simulink model "Copter_Plane_h2g_V10"  (R2020b)
settings: Solver=ode1  StartTime=0.0  StopTime=30  FixedStep=dt  RelTol=1e-3
values from neighbouring files (symbols this model uses):
  HD = 180/pi    (= 57.2957795131)    [mode_data.m]
undefined symbols (not defined in the file or in its folder): center_WP, GRAVITY_MSS, gyro_x, gyro_y, gyro_z, J, k_aileron, k_aileronL, k_aileronR, k_elevator, k_flap, k_rudder, m_kg, Newton, pid_vel_xy_derivative, pid_vel_xy_input, pid_vel_xy_integrator, pitch, POSCONTROL_ACC_Z_D, POSCONTROL_ACC_Z_P, POSCONTROL_VEL_XY_D, POSCONTROL_VEL_XY_P, pwm_out, pwm_tail, Raphson, roll, tail_tilt, Vehicle, vel_desired, yaw
libraries: shared6dofsys x3, sharedutil x3, simulink x1, aerolibasang x1
(part 2 of 3)

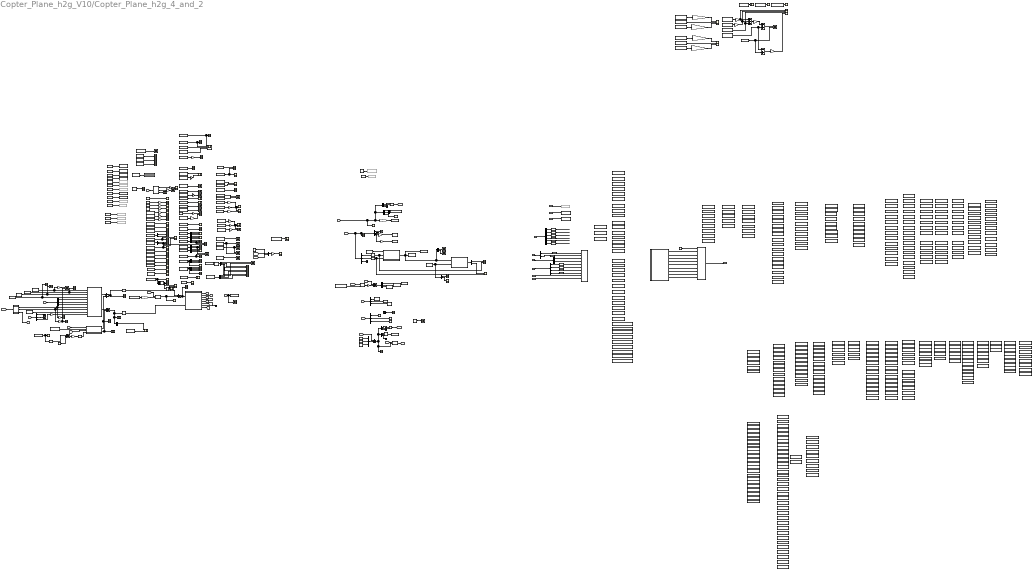
== system Copter_Plane_h2g_V10/Copter_Plane_h2g_4_and_2 ==
  CTRL_wp : Inport
  CTRL_remote_ct_st : Inport  Port=2  OutDataTypeStr=Bus: BUS_CTRL_remote_ct_st
  CTRL_dbg_param : Inport  Port=3  OutDataTypeStr=Bus: BUS_CTRL_dbg_param
  PathModeOut : Inport  Port=4  OutDataTypeStr=Bus: BUS_TASK_PATH_OutParam
  TASK_COMMON_OutParam : Inport  Port=5  OutDataTypeStr=Bus: BUS_TASK_COMMON_OutParam
  NAVI2CONTROL : Inport  Port=6  OutDataTypeStr=Bus: BUS_TO_CONTROL
  EAS_Algo : Inport  Port=7  OutDataTypeStr=Bus: BUS_AIRSPEED
  IMU : Inport  Port=8  OutDataTypeStr=Bus: BUS_IMU
  plane_mode_in : Inport  Port=9
  6DOF (Euler Angles)2 : Subsystem  AncestorBlock=shared6dof/6DOF (Euler Angles)  mask(6DOF EoM (Body Axis)){units=Metric (MKS), mtype=Fixed, rep=Euler Angles, xme_0=[0 0 -100], Vm_0=[10 -0 0], eul_0=[roll pitch yaw], pm_0=[gyro_x gyro_y gyro_z], mass_0=m_kg, mass_e=0.5, mass_f=2.0, inertia=J, inertia_e=eye(3), inertia_f=2*eye(3), k_quat=1.0, vre_flag=on, abi_flag=off, aMode=0, xme_statename='', Vm_statename='', eul_statename='', quat_statename='', pm_statename='', mass_statename=''}
      mask prompts: units "shared_aeroblks:sharedaeroblk6dofbody:block6DOFEoMBodyAxisParamUnits"; mtype "shared_aeroblks:sharedaeroblk6dofbody:block6DOFEoMBodyAxisParamMasstype"; rep "shared_aeroblks:sharedaeroblk6dofbody:block6DOFEoMBodyAxisParamRepresentation"; xme_0 "shared_aeroblks:sharedaeroblk6dofbody:block6DOFEoMBodyAxisParamInitialpositionininertialaxesXeYeZe"; Vm_0 "shared_aeroblks:sharedaeroblk6dofbody:block6DOFEoMBodyAxisParamInitialvelocityinbodyaxesUvw"; eul_0 "shared_aeroblks:sharedaeroblk6dofbody:block6DOFEoMBodyAxisParamInitialEulerorientationrollpitchyaw"; pm_0 "shared_aeroblks:sharedaeroblk6dofbody:block6DOFEoMBodyAxisParamInitialbodyrotationratespqr"; mass_0 "shared_aeroblks:sharedaeroblk6dofbody:block6DOFEoMBodyAxisParamInitialmass"; mass_e "shared_aeroblks:sharedaeroblk6dofbody:block6DOFEoMBodyAxisParamEmptymass"; mass_f "shared_aeroblks:sharedaeroblk6dofbody:block6DOFEoMBodyAxisParamFullmass"; inertia "shared_aeroblks:sharedaeroblk6dofbody:block6DOFEoMBodyAxisParamInertia"; inertia_e "shared_aeroblks:sharedaeroblk6dofbody:block6DOFEoMBodyAxisParamEmptyinertiamatrix"; inertia_f "shared_aeroblks:sharedaeroblk6dofbody:block6DOFEoMBodyAxisParamFullinertiamatrix"; k_quat "shared_aeroblks:sharedaeroblk6dofbody:block6DOFEoMBodyAxisParamGainforquaternionnormalization"; vre_flag "shared_aeroblks:sharedaeroblk6dofbody:block6DOFEoMBodyAxisParamIncludemassflowrelativevelocity"; abi_flag "shared_aeroblks:sharedaeroblk6dofbody:inertialAccelFlag"; xme_statename "shared_aeroblks:sharedaeroblk6dofbody:block6DOFEoMStateNamePosition"; Vm_statename "shared_aeroblks:sharedaeroblk6dofbody:block6DOFEoMStateNameVelocity"; eul_statename "shared_aeroblks:sharedaeroblk6dofbody:block6DOFEoMStateNameEulerAngles"; quat_statename "shared_aeroblks:sharedaeroblk6dofbody:block6DOFEoMStateNameQuaternions"; pm_statename "shared_aeroblks:sharedaeroblk6dofbody:block6DOFEoMStateNameRotationRates"; mass_statename "shared_aeroblks:sharedaeroblk6dofbody:block6DOFEoMStateNameMass"
      mask help: shared_aeroblks:sharedaeroblk6dofbody:block6DOFEoMBodyAxisDesc
      mask init:
      | if aerosharedtest(gcb)
      |     ports=aerosharedicon('shared6dofbody','icon');
      | else
      |     ports=sharedautoicon('shared6dofbody','icon');
      | end
      mask Help: eval('aerosharedhelp(''sixdof_euler_angles'')');
      mask TypeOptions units: shared_aeroblks:sharedaeroblk6dofbody:block6DOFEoMBodyAxisParamComboMetricMKS | shared_aeroblks:sharedaeroblk6dofbody:block6DOFEoMBodyAxisParamComboEnglishVelocityinfts | shared_aeroblks:sharedaeroblk6dofbody:block6DOFEoMBodyAxisParamComboEnglishVelocityinkts
      mask TypeOptions mtype: shared_aeroblks:sharedaeroblk6dofbody:block6DOFEoMBodyAxisParamComboFixed | shared_aeroblks:sharedaeroblk6dofbody:block6DOFEoMBodyAxisParamComboSimpleVariable | shared_aeroblks:sharedaeroblk6dofbody:block6DOFEoMBodyAxisParamComboCustomVariable
      mask Callback mtype:
      | if aerosharedtest(gcb) && builtin('license','test','aerospace_blockset')
      |     aerosharedicon('shared6dofbody');
      | else
      |     sharedautoicon('shared6dofbody');
      | end
      mask TypeOptions rep: shared_aeroblks:sharedaeroblk6dofbody:block6DOFEoMBodyAxisParamComboEulerAngles | shared_aeroblks:sharedaeroblk6dofbody:block6DOFEoMBodyAxisParamComboQuaternion
      mask Callback rep:
      | if aerosharedtest(gcb) && builtin('license','test','aerospace_blockset')
      |     aerosharedicon('shared6dofbody');
      | else
      |     sharedautoicon('shared6dofbody');
      | end
      mask DialogControl Container4 Prompt: shared_aeroblks:sharedaeroblk6dofbody:block6DOFEoMParamTab
      mask DialogControl units Prompt: Units:
      mask DialogControl mtype Prompt: Mass type:
      mask DialogControl rep Prompt: Representation:
      mask DialogControl xme_0 Prompt: Initial position in inertial axes [Xe,Ye,Ze]:
      mask DialogControl Vm_0 Prompt: Initial velocity in body axes [U,v,w]:
      mask DialogControl eul_0 Prompt: Initial Euler orientation [roll, pitch, yaw]:
      mask DialogControl pm_0 Prompt: Initial body rotation rates [p,q,r]:
      mask DialogControl mass_0 Prompt: Initial mass:
      mask DialogControl mass_e Prompt: Empty mass:
      mask DialogControl mass_f Prompt: Full mass:
      mask DialogControl inertia Prompt: Inertia:
      mask DialogControl inertia_e Prompt: Empty inertia matrix:
      mask DialogControl inertia_f Prompt: Full inertia matrix:
      mask DialogControl k_quat Prompt: Gain for quaternion normalization:
      mask DialogControl vre_flag Prompt: Include mass flow relative velocity
      mask DialogControl abi_flag Prompt: Include inertial acceleration
      mask DialogControl Container6 Prompt: shared_aeroblks:sharedaeroblk6dofbody:block6DOFEoMStateAttributesTab
      mask DialogControl Container7 Prompt: shared_aeroblks:sharedaeroblk6dofbody:block6DOFEoMStateNamesGroup
      mask DialogControl xme_statename Prompt: Position: e.g., {'Xe', 'Ye', 'Ze'}
      mask DialogControl Vm_statename Prompt: Velocity: e.g., {'U', 'v', 'w'}
      mask DialogControl eul_statename Prompt: Euler rotation angles: e.g., {'phi', 'theta', 'psi'}
      mask DialogControl quat_statename Prompt: Quaternion vector: e.g., {'qr', 'qi', 'qj', 'qk'}
      mask DialogControl pm_statename Prompt: Body rotation rates: e.g., {'p', 'q', 'r'}
      mask DialogControl mass_statename Prompt: Mass: e.g., 'mass'
      mask Display:
      | port_label(ports(1).type,ports(1).port,ports(1).txt,'texmode','on');
      | port_label(ports(2).type,ports(2).port,ports(2).txt,'texmode','on');
      | port_label(ports(3).type,ports(3).port,ports(3).txt,'texmode','on');
      | port_label(ports(4).type,ports(4).port,ports(4).txt,'texmode','on');
      | port_label(ports(5).type,ports(5).port,ports(5).txt,'texmode','on');
      | port_label(ports(6).type,ports(6).port,ports(6).txt,'texmode','on');
      | port_label(ports(7).type,ports(7).port,ports(7).txt,'texmode','on');
      | port_label(ports(8).type,ports(8).port,ports(8).txt,'texmode','on');
      | port_label(ports(9).type,ports(9).port,ports(9).txt,'texmode','on');
      | port_label(ports(10).type,ports(10).port,ports(10).txt,'texmode','on');
      | port_label(ports(11).type,ports(11).port,ports(11).txt,'texmode','on');
      | port_label(ports(12).type,ports(12).port,ports(12).txt,'texmode','on');
      | port_label(ports(13).type,ports(13).port,ports(13).txt,'texmode','on');
      | port_label(ports(14).type,ports(14).port,ports(14).txt,'texmode','on');
      | port_label(ports(15).type,ports(15).port,ports(15).txt,'texmode','on');
      | port_label(ports(16).type,ports(16).port,ports(16).txt,'texmode','on');
      | port_label(ports(17).type,ports(17).port,ports(17).txt,'texmode','on');
  AC_ATTITUDE_ACCEL_RP_CONTROLLER_MAX_RADSS1 : DataStoreMemory  DataStoreName=AC_ATTITUDE_ACCEL_RP_CONTROLLER_MAX_RADSS  ReadBeforeWriteMsg=warning  WriteAfterWriteMsg=warning  WriteAfterReadMsg=warning  InitialValue=AC_ATTITUDE_ACCEL_RP_CONTROLLER_MAX_RADSS  VectorParams1D=off  ShowAdditionalParam=off  OutDataTypeStr=double
  AC_ATTITUDE_ACCEL_RP_CONTROLLER_MIN_RADSS1 : DataStoreMemory  DataStoreName=AC_ATTITUDE_ACCEL_RP_CONTROLLER_MIN_RADSS  ReadBeforeWriteMsg=warning  WriteAfterWriteMsg=warning  WriteAfterReadMsg=warning  InitialValue=AC_ATTITUDE_ACCEL_RP_CONTROLLER_MIN_RADSS  VectorParams1D=off  ShowAdditionalParam=off  OutDataTypeStr=double
  AC_ATTITUDE_ACCEL_Y_CONTROLLER_MAX_RADSS1 : DataStoreMemory  DataStoreName=AC_ATTITUDE_ACCEL_Y_CONTROLLER_MAX_RADSS  ReadBeforeWriteMsg=warning  WriteAfterWriteMsg=warning  WriteAfterReadMsg=warning  InitialValue=AC_ATTITUDE_ACCEL_Y_CONTROLLER_MAX_RADSS  ShowAdditionalParam=off  OutDataTypeStr=double
  AC_ATTITUDE_ACCEL_Y_CONTROLLER_MIN_RADSS1 : DataStoreMemory  DataStoreName=AC_ATTITUDE_ACCEL_Y_CONTROLLER_MIN_RADSS  ReadBeforeWriteMsg=warning  WriteAfterWriteMsg=warning  WriteAfterReadMsg=warning  InitialValue=AC_ATTITUDE_ACCEL_Y_CONTROLLER_MIN_RADSS  VectorParams1D=off  ShowAdditionalParam=off  OutDataTypeStr=double
  AC_ATTITUDE_CONTROL_ANGLE_LIMIT_THROTTLE_MAX1 : DataStoreMemory  DataStoreName=AC_ATTITUDE_CONTROL_ANGLE_LIMIT_THROTTLE_MAX  ReadBeforeWriteMsg=warning  WriteAfterWriteMsg=warning  WriteAfterReadMsg=warning  InitialValue=AC_ATTITUDE_CONTROL_ANGLE_LIMIT_THROTTLE_MAX  VectorParams1D=off  ShowAdditionalParam=off  OutDataTypeStr=double
  AC_ATTITUDE_CONTROL_MAX1 : DataStoreMemory  DataStoreName=AC_ATTITUDE_CONTROL_MAX  ReadBeforeWriteMsg=warning  WriteAfterWriteMsg=warning  WriteAfterReadMsg=warning  InitialValue=AC_ATTITUDE_CONTROL_MAX  VectorParams1D=off  ShowAdditionalParam=off  OutDataTypeStr=double
  AC_ATTITUDE_THRUST_ERROR_ANGLE1 : DataStoreMemory  DataStoreName=AC_ATTITUDE_THRUST_ERROR_ANGLE  ReadBeforeWriteMsg=warning  WriteAfterWriteMsg=warning  WriteAfterReadMsg=warning  InitialValue=AC_ATTITUDE_THRUST_ERROR_ANGLE  ShowAdditionalParam=off  OutDataTypeStr=double
  AP_MOTORS_MATRIX_YAW_FACTOR_CCW1 : DataStoreMemory  DataStoreName=AP_MOTORS_MATRIX_YAW_FACTOR_CCW  ReadBeforeWriteMsg=warning  WriteAfterWriteMsg=warning  WriteAfterReadMsg=warning  InitialValue=AP_MOTORS_MATRIX_YAW_FACTOR_CCW  VectorParams1D=off  ShowAdditionalParam=off  OutDataTypeStr=double
  AP_MOTORS_MATRIX_YAW_FACTOR_CW1 : DataStoreMemory  DataStoreName=AP_MOTORS_MATRIX_YAW_FACTOR_CW  ReadBeforeWriteMsg=warning  WriteAfterWriteMsg=warning  WriteAfterReadMsg=warning  InitialValue=AP_MOTORS_MATRIX_YAW_FACTOR_CW  VectorParams1D=off  ShowAdditionalParam=off  OutDataTypeStr=double
  ATC_RAT_PIT_D1 : DataStoreMemory  DataStoreName=ATC_RAT_PIT_D  ReadBeforeWriteMsg=warning  WriteAfterWriteMsg=warning  WriteAfterReadMsg=warning  InitialValue=ATC_RAT_PIT_D  VectorParams1D=off  ShowAdditionalParam=off  OutDataTypeStr=double
  ATC_RAT_PIT_FF1 : DataStoreMemory  DataStoreName=ATC_RAT_PIT_FF  ReadBeforeWriteMsg=warning  WriteAfterWriteMsg=warning  WriteAfterReadMsg=warning  InitialValue=ATC_RAT_PIT_FF  VectorParams1D=off  ShowAdditionalParam=off  OutDataTypeStr=double
  ATC_RAT_PIT_FILT1 : DataStoreMemory  DataStoreName=ATC_RAT_PIT_FILT  ReadBeforeWriteMsg=warning  WriteAfterWriteMsg=warning  WriteAfterReadMsg=warning  InitialValue=ATC_RAT_PIT_FILT  VectorParams1D=off  ShowAdditionalParam=off  OutDataTypeStr=double
  ATC_RAT_PIT_I1 : DataStoreMemory  DataStoreName=ATC_RAT_PIT_I  ReadBeforeWriteMsg=warning  WriteAfterWriteMsg=warning  WriteAfterReadMsg=warning  InitialValue=ATC_RAT_PIT_I  VectorParams1D=off  ShowAdditionalParam=off  OutDataTypeStr=double
  ATC_RAT_PIT_IMAX1 : DataStoreMemory  DataStoreName=ATC_RAT_PIT_IMAX  ReadBeforeWriteMsg=warning  WriteAfterWriteMsg=warning  WriteAfterReadMsg=warning  InitialValue=ATC_RAT_PIT_IMAX  VectorParams1D=off  ShowAdditionalParam=off  OutDataTypeStr=double
  ATC_RAT_PIT_I_inint1 : DataStoreMemory  DataStoreName=ATC_RAT_PIT_I_inint  ReadBeforeWriteMsg=warning  WriteAfterWriteMsg=warning  WriteAfterReadMsg=warning  InitialValue=ATC_RAT_PIT_I_inint  VectorParams1D=off  ShowAdditionalParam=off  OutDataTypeStr=double
  ATC_RAT_PIT_P1 : DataStoreMemory  DataStoreName=ATC_RAT_PIT_P  ReadBeforeWriteMsg=warning  WriteAfterWriteMsg=warning  WriteAfterReadMsg=warning  InitialValue=ATC_RAT_PIT_P  VectorParams1D=off  ShowAdditionalParam=off  OutDataTypeStr=double
  ATC_RAT_RLL_D1 : DataStoreMemory  DataStoreName=ATC_RAT_RLL_D  ReadBeforeWriteMsg=warning  WriteAfterWriteMsg=warning  WriteAfterReadMsg=warning  InitialValue=ATC_RAT_RLL_D  VectorParams1D=off  ShowAdditionalParam=off  OutDataTypeStr=double
  ATC_RAT_RLL_FF1 : DataStoreMemory  DataStoreName=ATC_RAT_RLL_FF  ReadBeforeWriteMsg=warning  WriteAfterWriteMsg=warning  WriteAfterReadMsg=warning  InitialValue=ATC_RAT_RLL_FF  VectorParams1D=off  ShowAdditionalParam=off  OutDataTypeStr=double
  ATC_RAT_RLL_FILT1 : DataStoreMemory  DataStoreName=ATC_RAT_RLL_FILT  ReadBeforeWriteMsg=warning  WriteAfterWriteMsg=warning  WriteAfterReadMsg=warning  InitialValue=ATC_RAT_RLL_FILT  VectorParams1D=off  ShowAdditionalParam=off  OutDataTypeStr=double
  ATC_RAT_RLL_I1 : DataStoreMemory  DataStoreName=ATC_RAT_RLL_I  ReadBeforeWriteMsg=warning  WriteAfterWriteMsg=warning  WriteAfterReadMsg=warning  InitialValue=ATC_RAT_RLL_I  VectorParams1D=off  ShowAdditionalParam=off  OutDataTypeStr=double
  ATC_RAT_RLL_IMAX1 : DataStoreMemory  DataStoreName=ATC_RAT_RLL_IMAX  ReadBeforeWriteMsg=warning  WriteAfterWriteMsg=warning  WriteAfterReadMsg=warning  InitialValue=ATC_RAT_RLL_IMAX  VectorParams1D=off  ShowAdditionalParam=off  OutDataTypeStr=double
  ATC_RAT_RLL_I_inint1 : DataStoreMemory  DataStoreName=ATC_RAT_RLL_I_inint  ReadBeforeWriteMsg=warning  WriteAfterWriteMsg=warning  WriteAfterReadMsg=warning  InitialValue=ATC_RAT_RLL_I_inint  VectorParams1D=off  ShowAdditionalParam=off  OutDataTypeStr=double
  ATC_RAT_RLL_P1 : DataStoreMemory  DataStoreName=ATC_RAT_RLL_P  ReadBeforeWriteMsg=warning  WriteAfterWriteMsg=warning  WriteAfterReadMsg=warning  InitialValue=ATC_RAT_RLL_P  VectorParams1D=off  ShowAdditionalParam=off  OutDataTypeStr=double
  ATC_RAT_YAW_D1 : DataStoreMemory  DataStoreName=ATC_RAT_YAW_D  ReadBeforeWriteMsg=warning  WriteAfterWriteMsg=warning  WriteAfterReadMsg=warning  InitialValue=ATC_RAT_YAW_D  VectorParams1D=off  ShowAdditionalParam=off  OutDataTypeStr=double
  ATC_RAT_YAW_FF1 : DataStoreMemory  DataStoreName=ATC_RAT_YAW_FF  ReadBeforeWriteMsg=warning  WriteAfterWriteMsg=warning  WriteAfterReadMsg=warning  InitialValue=ATC_RAT_YAW_FF  VectorParams1D=off  ShowAdditionalParam=off  OutDataTypeStr=double
  ATC_RAT_YAW_FILT1 : DataStoreMemory  DataStoreName=ATC_RAT_YAW_FILT  ReadBeforeWriteMsg=warning  WriteAfterWriteMsg=warning  WriteAfterReadMsg=warning  InitialValue=ATC_RAT_YAW_FILT  VectorParams1D=off  ShowAdditionalParam=off  OutDataTypeStr=double
  ATC_RAT_YAW_I1 : DataStoreMemory  DataStoreName=ATC_RAT_YAW_I  ReadBeforeWriteMsg=warning  WriteAfterWriteMsg=warning  WriteAfterReadMsg=warning  InitialValue=ATC_RAT_YAW_I  VectorParams1D=off  ShowAdditionalParam=off  OutDataTypeStr=double
  ATC_RAT_YAW_IMAX1 : DataStoreMemory  DataStoreName=ATC_RAT_YAW_IMAX  ReadBeforeWriteMsg=warning  WriteAfterWriteMsg=warning  WriteAfterReadMsg=warning  InitialValue=ATC_RAT_YAW_IMAX  VectorParams1D=off  ShowAdditionalParam=off  OutDataTypeStr=double
  ATC_RAT_YAW_I_inint1 : DataStoreMemory  DataStoreName=ATC_RAT_YAW_I_inint  ReadBeforeWriteMsg=warning  WriteAfterWriteMsg=warning  WriteAfterReadMsg=warning  InitialValue=ATC_RAT_YAW_I_inint  VectorParams1D=off  ShowAdditionalParam=off  OutDataTypeStr=double
  ATC_RAT_YAW_P1 : DataStoreMemory  DataStoreName=ATC_RAT_YAW_P  ReadBeforeWriteMsg=warning  WriteAfterWriteMsg=warning  WriteAfterReadMsg=warning  InitialValue=ATC_RAT_YAW_P  VectorParams1D=off  ShowAdditionalParam=off  OutDataTypeStr=double
  Add : Sum  Inputs=+++
  Add{1..3,5,7} (5 alike) : Sum
  Add4 : Sum  Inputs=-+
  Add8 : Sum  Inputs=+-
  Atan3 : Trigonometry  Operator=atan2
  Atan4 : Trigonometry  Operator=atan2
  Bus Assignment : BusAssignment  AssignedSignals=k_aileron,k_elevator,k_rudder,k_aileronL,k_aileronR,tail_tilt,pwm_out,pwm_tail,k_flap
  Bus Selector : BusSelector  OutputSignals=curVelNED,curLLA
  Bus Selector1 : BusSelector  OutputSignals=pitchd,rolld,yawd,alt
  Bus Selector2 : BusSelector  OutputSignals=gyro_x,gyro_y,gyro_z,accel_x,accel_y,accel_z
  Bus Selector3 : BusSelector  OutputSignals=airspeed_indicate,EAS2TAS_Algo
  Constant : Constant  Value=0  OutDataTypeStr=Bus: BUS_CTRL_Sevro_pwm
  Constant1 : Constant  Value=0.3
  Constant{12..14,26,30,33,37,40..41} (9 alike) : Constant  Value=0
  Constant2 : Constant  Value=1000  VectorParams1D=off
  Constant25 : Constant  Value=500
  Constant27 : Constant  Value=10
  Constant28 : Constant  Value=500
  Constant29 : Constant  Value=000
  Constant31 : Constant  Value=[0;0]
  Constant32 : Constant  Value=0/HD
  Constant34 : Constant  Value=0.25
  Constant35 : Constant  Value=0.3
  Constant36 : Constant  Value=center_WP
  Constant38 : Constant  Value=center_WP
  Constant39 : Constant  Value=-30/HD
  Constant5 : Constant  Value=1.225
  Curr_sate : DataStoreMemory  DataStoreName=Curr_sate  ReadBeforeWriteMsg=warning  WriteAfterWriteMsg=warning  WriteAfterReadMsg=warning  InitialValue=Curr_sate  VectorParams1D=off  ShowAdditionalParam=off  OutDataTypeStr=Bus: BUS_CTRL_Curr_sate
  Data Store Read : DataStoreRead  DataStoreName=pitch_target
  Data Store Read1 : DataStoreRead  DataStoreName=pid_info_P_pitch
  Data Store Read10 : DataStoreRead  DataStoreName=pid_accel_z_integrator
  Data Store Read107 : DataStoreRead  DataStoreName=gyro_y
  Data Store Read108 : DataStoreRead  DataStoreName=curr_pos
  Data Store Read109 : DataStoreRead  DataStoreName=curr_alt
  Data Store Read11 : DataStoreRead  DataStoreName=pid_accel_z_input
  Data Store Read110 : DataStoreRead  DataStoreName=nav_bearing
  Data Store Read111 : DataStoreRead  DataStoreName=k_rudder
  Data Store Read112 : DataStoreRead  DataStoreName=k_aileron
  Data Store Read113 : DataStoreRead  DataStoreName=mode_L1
  Data Store Read114 : DataStoreRead  DataStoreName=k_throttle
  Data Store Read116 : DataStoreRead  DataStoreName=k_elevator
  Data Store Read117 : DataStoreRead  DataStoreName=roll
  Data Store Read118 : DataStoreRead  DataStoreName=pitch
  Data Store Read119 : DataStoreRead  DataStoreName=yaw
  Data Store Read12 : DataStoreRead  DataStoreName=pwm_out
  Data Store Read120 : DataStoreRead  DataStoreName=curr_vel
  Data Store Read121 : DataStoreRead  DataStoreName=z_accel_meas
  Data Store Read122 : DataStoreRead  DataStoreName=latAccDem
  Data Store Read123 : DataStoreRead  DataStoreName=accel_x
  Data Store Read124 : DataStoreRead  DataStoreName=accel_y
  Data Store Read125 : DataStoreRead  DataStoreName=accel_z
  Data Store Read126 : DataStoreRead  DataStoreName=pwm_out
  Data Store Read127 : DataStoreRead  DataStoreName=pos_target
  Data Store Read128 : DataStoreRead  DataStoreName=vel_target
  Data Store Read129 : DataStoreRead  DataStoreName=vel_desired
  Data Store Read13 : DataStoreRead  DataStoreName=thrust_rpyt_out
  Data Store Read130 : DataStoreRead  DataStoreName=accel_target
  Data Store Read131 : DataStoreRead  DataStoreName=accel_desired
  Data Store Read132 : DataStoreRead  DataStoreName=throttle_filter
  Data Store Read133 : DataStoreRead  DataStoreName=EAS_dem
  Data Store Read134 : DataStoreRead  DataStoreName=nav_pitch_cd
  Data Store Read135 : DataStoreRead  DataStoreName=aspeed
  Data Store Read136 : DataStoreRead  DataStoreName=nav_roll_cd
  Data Store Read137 : DataStoreRead  DataStoreName=k_rudder
  Data Store Read138 : DataStoreRead  DataStoreName=k_aileron
  Data Store Read139 : DataStoreRead  DataStoreName=k_throttle
  Data Store Read14 : DataStoreRead  DataStoreName=pitch_in
  Data Store Read140 : DataStoreRead  DataStoreName=k_elevator
  Data Store Read141 : DataStoreRead  DataStoreName=height
  Data Store Read142 : DataStoreRead  DataStoreName=Vz
  Data Store Read143 : DataStoreRead  DataStoreName=roll
  Data Store Read144 : DataStoreRead  DataStoreName=pid_vel_xy_input  DataStoreElements=pid_vel_xy_input(:,1)
  Data Store Read145 : DataStoreRead  DataStoreName=pid_vel_xy_integrator  DataStoreElements=pid_vel_xy_integrator(:,1)
  Data Store Read146 : DataStoreRead  DataStoreName=pid_vel_xy_derivative  DataStoreElements=pid_vel_xy_derivative(:,1)
  Data Store Read147 : DataStoreRead  DataStoreName=pid_vel_xy_input  DataStoreElements=pid_vel_xy_input(:,2)
  Data Store Read148 : DataStoreRead  DataStoreName=pid_vel_xy_integrator  DataStoreElements=pid_vel_xy_integrator(:,2)
  Data Store Read149 : DataStoreRead  DataStoreName=pid_vel_xy_derivative  DataStoreElements=pid_vel_xy_derivative(:,2)
  Data Store Read15 : DataStoreRead  DataStoreName=k_flap
  Data Store Read150 : DataStoreRead  DataStoreName=pid_info_I_pitch
  Data Store Read151 : DataStoreRead  DataStoreName=last_out_pitch
  Data Store Read16 : DataStoreRead  DataStoreName=aspeed
  Data Store Read166 : DataStoreRead  DataStoreName=throttle_hover
  Data Store Read167 : DataStoreRead  DataStoreName=throttle_in
  Data Store Read17 : DataStoreRead  DataStoreName=pwm_out
  Data Store Read18 : DataStoreRead  DataStoreName=plane_mode
  Data Store Read2 : DataStoreRead  DataStoreName=k_flap_Land
  Data Store Read3 : DataStoreRead  DataStoreName=k_flap_TakeOff
  Data Store Read34 : DataStoreRead  DataStoreName=hgt_rate_dem
  Data Store Read36 : DataStoreRead  DataStoreName=nav_roll_cd
  Data Store Read37 : DataStoreRead  DataStoreName=throttle_dem
  Data Store Read38 : DataStoreRead  DataStoreName=pitch_dem
  Data Store Read39 : DataStoreRead  DataStoreName=nav_pitch_cd
  Data Store Read4 : DataStoreRead  DataStoreName=rate_roll_pid_integrator
  Data Store Read40 : DataStoreRead  DataStoreName=pitch
  Data Store Read41 : DataStoreRead  DataStoreName=pid_info_desired_pitch
  Data Store Read42 : DataStoreRead  DataStoreName=pid_info_actual_pitch
  Data Store Read43 : DataStoreRead  DataStoreName=hgt_dem_adj
  Data Store Read44 : DataStoreRead  DataStoreName=height
  Data Store Read45 : DataStoreRead  DataStoreName=hgt_dem_adj
  Data Store Read46 : DataStoreRead  DataStoreName=Vz
  Data Store Read48 : DataStoreRead  DataStoreName=thrust_rpyt_out
  Data Store Read5 : DataStoreRead  DataStoreName=rate_pitch_pid_integrator
  Data Store Read50 : DataStoreRead  DataStoreName=pitch_in
  Data Store Read53 : DataStoreRead  DataStoreName=pitch_target
  Data Store Read54 : DataStoreRead  DataStoreName=roll_target
  Data Store Read55 : DataStoreRead  DataStoreName=target_yaw_rate
  Data Store Read56 : DataStoreRead  DataStoreName=mode
  Data Store Read57 : DataStoreRead  DataStoreName=tail_tilt
  Data Store Read58 : DataStoreRead  DataStoreName=tail_tilt
  Data Store Read59 : DataStoreRead  DataStoreName=accel_last_z_cms
  Data Store Read6 : DataStoreRead  DataStoreName=pwm_tail
  Data Store Read60 : DataStoreRead  DataStoreName=PathModeOut_sl  DataStoreElements=PathModeOut_sl.flightTaskMode
  Data Store Read62 : DataStoreRead  DataStoreName=pitch_in
  Data Store Read63 : DataStoreRead  DataStoreName=roll_in
  Data Store Read64 : DataStoreRead  DataStoreName=yaw_in
  Data Store Read65 : DataStoreRead  DataStoreName=groundspeed_vector
  Data Store Read66 : DataStoreRead  DataStoreName=yaw
  Data Store Read67 : DataStoreRead  DataStoreName=vel_forward_last_pct
  Data Store Read68 : DataStoreRead  DataStoreName=gyro_x
  Data Store Read69 : DataStoreRead  DataStoreName=tail_tilt
  Data Store Read7 : DataStoreRead  DataStoreName=pitch
  Data Store Read70 : DataStoreRead  DataStoreName=rate_pitch_pid_integrator
  Data Store Read71 : DataStoreRead  DataStoreName=throttle_in
  Data Store Read74 : DataStoreRead  DataStoreName=gyro_z
  Data Store Read79 : DataStoreRead  DataStoreName=pid_info_D_pitch
  Data Store Read8 : DataStoreRead  DataStoreName=rate_yaw_pid_integrator
  Data Store Read83 : DataStoreRead  DataStoreName=gyro_y
  Data Store Read9 : DataStoreRead  DataStoreName=pid_accel_z_derivative
  Data Store Write : DataStoreWrite  DataStoreName=algo_remote_ct_st
  Data Store Write1 : DataStoreWrite  DataStoreName=algo_dbg_param
  Data Store Write2 : DataStoreWrite  DataStoreName=Curr_sate  DataStoreElements=Curr_sate.EAS_Algo#Curr_sate.EAS2TAS_Algo#Curr_sate.curVelNED(:,:)#Curr_sate.curLLA(:,:)#Curr_sate.pitchd#Curr_sate.rolld#Curr_sate.yawd#Curr_sate.NAV_alt#Curr_sate.PathModeOut#Curr_sate.wp_in(:,:)
  Data Store Write3 : DataStoreWrite  Commented=on  DataStoreName=plane_mode
  Data Store Write31 : DataStoreWrite  DataStoreName=throttle_in
  Data Store Write32 : DataStoreWrite  DataStoreName=aspeed
  Data Store Write33 : DataStoreWrite  Commented=on  DataStoreName=tail_tilt
  Data Store Write34 : DataStoreWrite  DataStoreName=climb_rate_cms
  Data Store Write35 : DataStoreWrite  DataStoreName=mode
  Data Store Write36 : DataStoreWrite  DataStoreName=vel_desired  DataStoreElements=vel_desired(1,1:2)
  Data Store Write37 : DataStoreWrite  Commented=on  DataStoreName=throttle_dem
  Data Store Write38 : DataStoreWrite  DataStoreName=pitch
  Data Store Write39 : DataStoreWrite  DataStoreName=accel_y
  Data Store Write4 : DataStoreWrite  Commented=on  DataStoreName=k_throttle
  Data Store Write40 : DataStoreWrite  DataStoreName=accel_x
  Data Store Write41 : DataStoreWrite  DataStoreName=current_loc
  Data Store Write42 : DataStoreWrite  DataStoreName=groundspeed_vector
  Data Store Write43 : DataStoreWrite  Commented=on  DataStoreName=pitch_target
  Data Store Write44 : DataStoreWrite  DataStoreName=accel_z
  Data Store Write45 : DataStoreWrite  Commented=on  DataStoreName=pitch_dem
  Data Store Write46 : DataStoreWrite  Commented=on  DataStoreName=pitch_dem
  Data Store Write47 : DataStoreWrite  Commented=on  DataStoreName=latAccDem
  Data Store Write48 : DataStoreWrite  Commented=on  DataStoreName=latAccDem
  Data Store Write49 : DataStoreWrite  DataStoreName=Vz
  Data Store Write50 : DataStoreWrite  DataStoreName=height
  Data Store Write51 : DataStoreWrite  DataStoreName=roll
  Data Store Write52 : DataStoreWrite  DataStoreName=yaw
  Data Store Write53 : DataStoreWrite  DataStoreName=roll_target_pilot
  Data Store Write54 : DataStoreWrite  Commented=on  DataStoreName=roll_target
  Data Store Write55 : DataStoreWrite  DataStoreName=pitch_target_pilot
  Data Store Write56 : DataStoreWrite  DataStoreName=gyro_x
  Data Store Write57 : DataStoreWrite  DataStoreName=gyro_y
  Data Store Write58 : DataStoreWrite  DataStoreName=gyro_z
  Data Store Write59 : DataStoreWrite  DataStoreName=curr_alt
  Data Store Write60 : DataStoreWrite  Commented=on  DataStoreName=target_yaw_rate
  Data Store Write61 : DataStoreWrite  DataStoreName=curr_vel
  Data Type Conversion{,1..11} (12 alike) : DataTypeConversion
  Delay{4..7} (4 alike) : Delay  DelayLength=1  InitialCondition=0
  Demux{,10,12..13,16,19..23,37..41,44,46..47} (18 alike) : Demux  Outputs=3
  Demux{1..2,14..15} (4 alike) : Demux
  Demux{9,36,42..43,45} (5 alike) : Demux  Outputs=2
  Derivative1 : Derivative
  Display1 : Display
  EAS2TAS1 : DataStoreMemory  DataStoreName=EAS2TAS  ReadBeforeWriteMsg=warning  WriteAfterWriteMsg=warning  WriteAfterReadMsg=warning  InitialValue=EAS2TAS  VectorParams1D=off  ShowAdditionalParam=off  OutDataTypeStr=double
  EAS_dem1 : DataStoreMemory  DataStoreName=EAS_dem  ReadBeforeWriteMsg=warning  WriteAfterWriteMsg=warning  WriteAfterReadMsg=warning  InitialValue=EAS_dem  VectorParams1D=off  ShowAdditionalParam=off  OutDataTypeStr=double
  EAS_dem_cm1 : DataStoreMemory  DataStoreName=EAS_dem_cm  ReadBeforeWriteMsg=warning  WriteAfterWriteMsg=warning  WriteAfterReadMsg=warning  InitialValue=EAS_dem_cm  VectorParams1D=off  ShowAdditionalParam=off  OutDataTypeStr=double
  Fix2Rotor_delay_s : DataStoreMemory  DataStoreName=Fix2Rotor_delay_s  ReadBeforeWriteMsg=warning  WriteAfterWriteMsg=warning  WriteAfterReadMsg=warning  InitialValue=Fix2Rotor_delay_s  VectorParams1D=off  ShowAdditionalParam=off  OutDataTypeStr=double
  GRAVITY_MSS1 : DataStoreMemory  DataStoreName=GRAVITY_MSS  ReadBeforeWriteMsg=warning  WriteAfterWriteMsg=warning  WriteAfterReadMsg=warning  InitialValue=GRAVITY_MSS  VectorParams1D=off  ShowAdditionalParam=off  OutDataTypeStr=double
  Gain : Gain  Gain=1/1000
  Gain{1,3,14,31..38,40..41,43,48..49} (16 alike) : Gain  Gain=HD
  Gain2 : Gain  Gain=1/100
  Gain{26..29} (4 alike) : Gain  Gain=-1
  Gain30 : Gain  Gain=1/100
  Gain{39,42,46..47} (4 alike) : Gain  Gain=0.01
  Gain44 : Gain  Gain=-100
  Gain45 : Gain  Gain=[100 100 -100]
  Gain72 : Gain  Gain=POSCONTROL_ACC_Z_D
  Gain76 : Gain  Gain=POSCONTROL_VEL_XY_P
  Gain77 : Gain  Gain=POSCONTROL_VEL_XY_D
  Gain78 : Gain  Gain=POSCONTROL_VEL_XY_P
  Gain79 : Gain  Gain=POSCONTROL_VEL_XY_D
  Gain83 : Gain  Gain=POSCONTROL_ACC_Z_P
  Gain84 : Gain  Gain=0.001
  Gain85 : Gain  Gain=1000
  Gravity in Earth Axes2 : Gain  Gain=m_kg  SaturateOnIntegerOverflow=on  OutDataTypeStr=Inherit: Same as input  ParamDataTypeStr=Inherit: Same as input
  HD1 : DataStoreMemory  DataStoreName=HD  ReadBeforeWriteMsg=warning  WriteAfterWriteMsg=warning  WriteAfterReadMsg=warning  InitialValue=HD  ShowAdditionalParam=off  OutDataTypeStr=double
  Hypot2 : Math  Operator=hypot  SaturateOnIntegerOverflow=on
  Hypot3 : Math  Operator=hypot  SaturateOnIntegerOverflow=on
  "Incidence, Sideslip & Airspeed2" : Subsystem  AncestorBlock=aerolibasang/Incidence, Sideslip, & Airspeed  mask(Incidence,Sideslip,&Airspeed){}
      mask help: aeroblks:aeroblkasang:blockIncidenceSideslipAirspeedDesc
      mask init:
      | aeroicon('aeroblk');
      mask Help: eval('asbhelp(''incidence_sideslip_and_airspeed'')');
      mask Display:
      | port_label('input',1,'V_b','texmode','on');
      | port_label('output',1,'\alpha','texmode','on');
      | port_label('output',2,'\beta','texmode','on');
      | port_label('output',3,'V','texmode','on');
  "Incidence, Sideslip & Airspeed3" : aerolibasang/Incidence, Sideslip, & Airspeed
  Inertial to Body4 : Product  Multiplication=Matrix(*)  InputSameDT=on  SaturateOnIntegerOverflow=on  OutDataTypeStr=Inherit: Same as first input
  Inertial to Body5 : Product  Multiplication=Matrix(*)  InputSameDT=on  SaturateOnIntegerOverflow=on  OutDataTypeStr=Inherit: Same as first input
  Inertial to Body6 : Product  Multiplication=Matrix(*)  InputSameDT=on  SaturateOnIntegerOverflow=on  OutDataTypeStr=Inherit: Same as first input
  K_A_yaw1 : DataStoreMemory  DataStoreName=K_A_yaw  ReadBeforeWriteMsg=warning  WriteAfterWriteMsg=warning  WriteAfterReadMsg=warning  InitialValue=K_A_yaw  ShowAdditionalParam=off  OutDataTypeStr=double
  K_D_last_yaw1 : DataStoreMemory  DataStoreName=K_D_last_yaw  ReadBeforeWriteMsg=warning  WriteAfterWriteMsg=warning  WriteAfterReadMsg=warning  InitialValue=K_D_last_yaw  ShowAdditionalParam=off  OutDataTypeStr=double
  K_D_yaw1 : DataStoreMemory  DataStoreName=K_D_yaw  ReadBeforeWriteMsg=warning  WriteAfterWriteMsg=warning  WriteAfterReadMsg=warning  InitialValue=K_D_yaw  ShowAdditionalParam=off  OutDataTypeStr=double
  K_FF_yaw1 : DataStoreMemory  DataStoreName=K_FF_yaw  ReadBeforeWriteMsg=warning  WriteAfterWriteMsg=warning  WriteAfterReadMsg=warning  InitialValue=K_FF_yaw  ShowAdditionalParam=off  OutDataTypeStr=double
  K_FF_yaw_inint1 : DataStoreMemory  DataStoreName=K_FF_yaw_inint  ReadBeforeWriteMsg=warning  WriteAfterWriteMsg=warning  WriteAfterReadMsg=warning  InitialValue=K_FF_yaw_inint  VectorParams1D=off  ShowAdditionalParam=off  OutDataTypeStr=double
  K_I_yaw1 : DataStoreMemory  DataStoreName=K_I_yaw  ReadBeforeWriteMsg=warning  WriteAfterWriteMsg=warning  WriteAfterReadMsg=warning  InitialValue=K_I_yaw  ShowAdditionalParam=off  OutDataTypeStr=double
  Kx1 : DataStoreMemory  DataStoreName=Kx  ReadBeforeWriteMsg=warning  WriteAfterWriteMsg=warning  WriteAfterReadMsg=warning  InitialValue=Kx  VectorParams1D=off  ShowAdditionalParam=off  OutDataTypeStr=double
  L1_damping1 : DataStoreMemory  DataStoreName=L1_damping  ReadBeforeWriteMsg=warning  WriteAfterWriteMsg=warning  WriteAfterReadMsg=warning  InitialValue=L1_damping  VectorParams1D=off  ShowAdditionalParam=off  OutDataTypeStr=double
  L1_dist1 : DataStoreMemory  DataStoreName=L1_dist  ReadBeforeWriteMsg=warning  WriteAfterWriteMsg=warning  WriteAfterReadMsg=warning  InitialValue=L1_dist  VectorParams1D=off  ShowAdditionalParam=off  OutDataTypeStr=double
  L1_period1 : DataStoreMemory  DataStoreName=L1_period  ReadBeforeWriteMsg=warning  WriteAfterWriteMsg=warning  WriteAfterReadMsg=warning  InitialValue=L1_period  VectorParams1D=off  ShowAdditionalParam=off  OutDataTypeStr=double
  L1_radius1 : DataStoreMemory  DataStoreName=L1_radius  ReadBeforeWriteMsg=warning  WriteAfterWriteMsg=warning  WriteAfterReadMsg=warning  InitialValue=L1_radius  VectorParams1D=off  ShowAdditionalParam=off  OutDataTypeStr=double
  L1_xtrack_i1 : DataStoreMemory  DataStoreName=L1_xtrack_i  ReadBeforeWriteMsg=warning  WriteAfterWriteMsg=warning  WriteAfterReadMsg=warning  InitialValue=L1_xtrack_i  VectorParams1D=off  ShowAdditionalParam=off  OutDataTypeStr=double
  L1_xtrack_i_gain1 : DataStoreMemory  DataStoreName=L1_xtrack_i_gain  ReadBeforeWriteMsg=warning  WriteAfterWriteMsg=warning  WriteAfterReadMsg=warning  InitialValue=L1_xtrack_i_gain  VectorParams1D=off  ShowAdditionalParam=off  OutDataTypeStr=double
  L1_xtrack_i_gain_prev1 : DataStoreMemory  DataStoreName=L1_xtrack_i_gain_prev  ReadBeforeWriteMsg=warning  WriteAfterWriteMsg=warning  WriteAfterReadMsg=warning  InitialValue=L1_xtrack_i_gain_prev  VectorParams1D=off  ShowAdditionalParam=off  OutDataTypeStr=double
  LOCATION_SCALING_FACTOR1 : DataStoreMemory  DataStoreName=LOCATION_SCALING_FACTOR  ReadBeforeWriteMsg=warning  WriteAfterWriteMsg=warning  WriteAfterReadMsg=warning  InitialValue=LOCATION_SCALING_FACTOR  VectorParams1D=off  ShowAdditionalParam=off  OutDataTypeStr=double
  LOCATION_SCALING_FACTOR_INV1 : DataStoreMemory  DataStoreName=LOCATION_SCALING_FACTOR_INV  ReadBeforeWriteMsg=warning  WriteAfterWriteMsg=warning  WriteAfterReadMsg=warning  InitialValue=LOCATION_SCALING_FACTOR_INV  VectorParams1D=off  ShowAdditionalParam=off  OutDataTypeStr=double
  Location_offset1 : MATLAB Function  TreatAsAtomicUnit=on
  MATLAB Function : MATLAB Function  TreatAsAtomicUnit=on
  MATLAB Function1 : MATLAB Function  TreatAsAtomicUnit=on
  Mux3 : Mux  Inputs=2
  Mux4 : Mux  Inputs=3
  Mux5 : Mux  Inputs=3
  PITCHmaxf1 : DataStoreMemory  DataStoreName=PITCHmaxf  ReadBeforeWriteMsg=warning  WriteAfterWriteMsg=warning  WriteAfterReadMsg=warning  InitialValue=PITCHmaxf  VectorParams1D=off  ShowAdditionalParam=off  OutDataTypeStr=double
  PITCHminf1 : DataStoreMemory  DataStoreName=PITCHminf  ReadBeforeWriteMsg=warning  WriteAfterWriteMsg=warning  WriteAfterReadMsg=warning  InitialValue=PITCHminf  VectorParams1D=off  ShowAdditionalParam=off  OutDataTypeStr=double
  POSCONTROL_ACCELERATION_MIN1 : DataStoreMemory  DataStoreName=POSCONTROL_ACCELERATION_MIN  ReadBeforeWriteMsg=warning  WriteAfterWriteMsg=warning  WriteAfterReadMsg=warning  InitialValue=POSCONTROL_ACCELERATION_MIN  ShowAdditionalParam=off  OutDataTypeStr=double
  POSCONTROL_ACCEL_FILTER_HZ1 : DataStoreMemory  DataStoreName=POSCONTROL_ACCEL_FILTER_HZ  ReadBeforeWriteMsg=warning  WriteAfterWriteMsg=warning  WriteAfterReadMsg=warning  InitialValue=POSCONTROL_ACCEL_FILTER_HZ  VectorParams1D=off  ShowAdditionalParam=off  OutDataTypeStr=double
  POSCONTROL_ACCEL_XY1 : DataStoreMemory  DataStoreName=POSCONTROL_ACCEL_XY  ReadBeforeWriteMsg=warning  WriteAfterWriteMsg=warning  WriteAfterReadMsg=warning  InitialValue=POSCONTROL_ACCEL_XY  VectorParams1D=off  ShowAdditionalParam=off  OutDataTypeStr=double
  POSCONTROL_ACCEL_XY_MAX1 : DataStoreMemory  DataStoreName=POSCONTROL_ACCEL_XY_MAX  ReadBeforeWriteMsg=warning  WriteAfterWriteMsg=warning  WriteAfterReadMsg=warning  InitialValue=POSCONTROL_ACCEL_XY_MAX  VectorParams1D=off  ShowAdditionalParam=off  OutDataTypeStr=double
  POSCONTROL_ACCEL_Z1 : DataStoreMemory  DataStoreName=POSCONTROL_ACCEL_Z  ReadBeforeWriteMsg=warning  WriteAfterWriteMsg=warning  WriteAfterReadMsg=warning  InitialValue=POSCONTROL_ACCEL_Z  ShowAdditionalParam=off  OutDataTypeStr=double
  POSCONTROL_ACC_Z_D1 : DataStoreMemory  DataStoreName=POSCONTROL_ACC_Z_D  ReadBeforeWriteMsg=warning  WriteAfterWriteMsg=warning  WriteAfterReadMsg=warning  InitialValue=POSCONTROL_ACC_Z_D  VectorParams1D=off  ShowAdditionalParam=off  OutDataTypeStr=double
  POSCONTROL_ACC_Z_FILT_HZ1 : DataStoreMemory  DataStoreName=POSCONTROL_ACC_Z_FILT_HZ  ReadBeforeWriteMsg=warning  WriteAfterWriteMsg=warning  WriteAfterReadMsg=warning  InitialValue=POSCONTROL_ACC_Z_FILT_HZ  VectorParams1D=off  ShowAdditionalParam=off  OutDataTypeStr=double
  POSCONTROL_ACC_Z_FILT_HZ_c2p1 : DataStoreMemory  DataStoreName=POSCONTROL_ACC_Z_FILT_HZ_c2p  ReadBeforeWriteMsg=warning  WriteAfterWriteMsg=warning  WriteAfterReadMsg=warning  InitialValue=POSCONTROL_ACC_Z_FILT_HZ_c2p  VectorParams1D=off  ShowAdditionalParam=off  OutDataTypeStr=double
  POSCONTROL_ACC_Z_FILT_HZ_inint1 : DataStoreMemory  DataStoreName=POSCONTROL_ACC_Z_FILT_HZ_inint  ReadBeforeWriteMsg=warning  WriteAfterWriteMsg=warning  WriteAfterReadMsg=warning  InitialValue=POSCONTROL_ACC_Z_FILT_HZ_inint  VectorParams1D=off  ShowAdditionalParam=off  OutDataTypeStr=double
  POSCONTROL_ACC_Z_I1 : DataStoreMemory  DataStoreName=POSCONTROL_ACC_Z_I  ReadBeforeWriteMsg=warning  WriteAfterWriteMsg=warning  WriteAfterReadMsg=warning  InitialValue=POSCONTROL_ACC_Z_I  VectorParams1D=off  ShowAdditionalParam=off  OutDataTypeStr=double
  POSCONTROL_ACC_Z_IMAX1 : DataStoreMemory  DataStoreName=POSCONTROL_ACC_Z_IMAX  ReadBeforeWriteMsg=warning  WriteAfterWriteMsg=warning  WriteAfterReadMsg=warning  InitialValue=POSCONTROL_ACC_Z_IMAX  VectorParams1D=off  ShowAdditionalParam=off  OutDataTypeStr=double
  POSCONTROL_ACC_Z_I_inint1 : DataStoreMemory  DataStoreName=POSCONTROL_ACC_Z_I_inint  ReadBeforeWriteMsg=warning  WriteAfterWriteMsg=warning  WriteAfterReadMsg=warning  InitialValue=POSCONTROL_ACC_Z_I_inint  VectorParams1D=off  ShowAdditionalParam=off  OutDataTypeStr=double
  POSCONTROL_ACC_Z_P1 : DataStoreMemory  DataStoreName=POSCONTROL_ACC_Z_P  ReadBeforeWriteMsg=warning  WriteAfterWriteMsg=warning  WriteAfterReadMsg=warning  InitialValue=POSCONTROL_ACC_Z_P  VectorParams1D=off  ShowAdditionalParam=off  OutDataTypeStr=double
  POSCONTROL_JERK_RATIO1 : DataStoreMemory  DataStoreName=POSCONTROL_JERK_RATIO  ReadBeforeWriteMsg=warning  WriteAfterWriteMsg=warning  WriteAfterReadMsg=warning  InitialValue=POSCONTROL_JERK_RATIO  VectorParams1D=off  ShowAdditionalParam=off  OutDataTypeStr=double
  POSCONTROL_LEASH_LENGTH_MIN1 : DataStoreMemory  DataStoreName=POSCONTROL_LEASH_LENGTH_MIN  ReadBeforeWriteMsg=warning  WriteAfterWriteMsg=warning  WriteAfterReadMsg=warning  InitialValue=POSCONTROL_LEASH_LENGTH_MIN  VectorParams1D=off  ShowAdditionalParam=off  OutDataTypeStr=double
  POSCONTROL_OVERSPEED_GAIN_Z1 : DataStoreMemory  DataStoreName=POSCONTROL_OVERSPEED_GAIN_Z  ReadBeforeWriteMsg=warning  WriteAfterWriteMsg=warning  WriteAfterReadMsg=warning  InitialValue=POSCONTROL_OVERSPEED_GAIN_Z  VectorParams1D=off  ShowAdditionalParam=off  OutDataTypeStr=double
  POSCONTROL_POS_XY_P1 : DataStoreMemory  DataStoreName=POSCONTROL_POS_XY_P  ReadBeforeWriteMsg=warning  WriteAfterWriteMsg=warning  WriteAfterReadMsg=warning  InitialValue=POSCONTROL_POS_XY_P  VectorParams1D=off  ShowAdditionalParam=off  OutDataTypeStr=double
  POSCONTROL_POS_Z_P1 : DataStoreMemory  DataStoreName=POSCONTROL_POS_Z_P  ReadBeforeWriteMsg=warning  WriteAfterWriteMsg=warning  WriteAfterReadMsg=warning  InitialValue=POSCONTROL_POS_Z_P  VectorParams1D=off  ShowAdditionalParam=off  OutDataTypeStr=double
  POSCONTROL_SPEED1 : DataStoreMemory  DataStoreName=POSCONTROL_SPEED  ReadBeforeWriteMsg=warning  WriteAfterWriteMsg=warning  WriteAfterReadMsg=warning  InitialValue=POSCONTROL_SPEED  ShowAdditionalParam=off  OutDataTypeStr=double
  POSCONTROL_SPEED_DOWN1 : DataStoreMemory  DataStoreName=POSCONTROL_SPEED_DOWN  ReadBeforeWriteMsg=warning  WriteAfterWriteMsg=warning  WriteAfterReadMsg=warning  InitialValue=POSCONTROL_SPEED_DOWN  ShowAdditionalParam=off  OutDataTypeStr=double
  POSCONTROL_SPEED_UP1 : DataStoreMemory  DataStoreName=POSCONTROL_SPEED_UP  ReadBeforeWriteMsg=warning  WriteAfterWriteMsg=warning  WriteAfterReadMsg=warning  InitialValue=POSCONTROL_SPEED_UP  ShowAdditionalParam=off  OutDataTypeStr=double
  POSCONTROL_STOPPING_DIST_DOWN_MAX1 : DataStoreMemory  DataStoreName=POSCONTROL_STOPPING_DIST_DOWN_MAX  ReadBeforeWriteMsg=warning  WriteAfterWriteMsg=warning  WriteAfterReadMsg=warning  InitialValue=POSCONTROL_STOPPING_DIST_DOWN_MAX  VectorParams1D=off  ShowAdditionalParam=off  OutDataTypeStr=double
  POSCONTROL_STOPPING_DIST_UP_MAX1 : DataStoreMemory  DataStoreName=POSCONTROL_STOPPING_DIST_UP_MAX  ReadBeforeWriteMsg=warning  WriteAfterWriteMsg=warning  WriteAfterReadMsg=warning  InitialValue=POSCONTROL_STOPPING_DIST_UP_MAX  VectorParams1D=off  ShowAdditionalParam=off  OutDataTypeStr=double
  POSCONTROL_THROTTLE_CUTOFF_FREQ1 : DataStoreMemory  DataStoreName=POSCONTROL_THROTTLE_CUTOFF_FREQ  ReadBeforeWriteMsg=warning  WriteAfterWriteMsg=warning  WriteAfterReadMsg=warning  InitialValue=POSCONTROL_THROTTLE_CUTOFF_FREQ  VectorParams1D=off  ShowAdditionalParam=off  OutDataTypeStr=double
  POSCONTROL_THROTTLE_CUTOFF_FREQ_inint : DataStoreMemory  DataStoreName=POSCONTROL_THROTTLE_CUTOFF_FREQ_inint  ReadBeforeWriteMsg=warning  WriteAfterWriteMsg=warning  WriteAfterReadMsg=warning  InitialValue=POSCONTROL_THROTTLE_CUTOFF_FREQ_inint  VectorParams1D=off  ShowAdditionalParam=off  OutDataTypeStr=double
  POSCONTROL_THROTTLE_CUTOFF_FREQ_p2c : DataStoreMemory  DataStoreName=POSCONTROL_THROTTLE_CUTOFF_FREQ_p2c  ReadBeforeWriteMsg=warning  WriteAfterWriteMsg=warning  WriteAfterReadMsg=warning  InitialValue=POSCONTROL_THROTTLE_CUTOFF_FREQ_p2c  VectorParams1D=off  ShowAdditionalParam=off  OutDataTypeStr=double
  POSCONTROL_VEL_ERROR_CUTOFF_FREQ1 : DataStoreMemory  DataStoreName=POSCONTROL_VEL_ERROR_CUTOFF_FREQ  ReadBeforeWriteMsg=warning  WriteAfterWriteMsg=warning  WriteAfterReadMsg=warning  InitialValue=POSCONTROL_VEL_ERROR_CUTOFF_FREQ  VectorParams1D=off  ShowAdditionalParam=off  OutDataTypeStr=double
  POSCONTROL_VEL_XY_D1 : DataStoreMemory  DataStoreName=POSCONTROL_VEL_XY_D  ReadBeforeWriteMsg=warning  WriteAfterWriteMsg=warning  WriteAfterReadMsg=warning  InitialValue=POSCONTROL_VEL_XY_D  VectorParams1D=off  ShowAdditionalParam=off  OutDataTypeStr=double
  POSCONTROL_VEL_XY_FILT_D_HZ1 : DataStoreMemory  DataStoreName=POSCONTROL_VEL_XY_FILT_D_HZ  ReadBeforeWriteMsg=warning  WriteAfterWriteMsg=warning  WriteAfterReadMsg=warning  InitialValue=POSCONTROL_VEL_XY_FILT_D_HZ  VectorParams1D=off  ShowAdditionalParam=off  OutDataTypeStr=double
  POSCONTROL_VEL_XY_FILT_HZ1 : DataStoreMemory  DataStoreName=POSCONTROL_VEL_XY_FILT_HZ  ReadBeforeWriteMsg=warning  WriteAfterWriteMsg=warning  WriteAfterReadMsg=warning  InitialValue=POSCONTROL_VEL_XY_FILT_HZ  VectorParams1D=off  ShowAdditionalParam=off  OutDataTypeStr=double
  POSCONTROL_VEL_XY_I1 : DataStoreMemory  DataStoreName=POSCONTROL_VEL_XY_I  ReadBeforeWriteMsg=warning  WriteAfterWriteMsg=warning  WriteAfterReadMsg=warning  InitialValue=POSCONTROL_VEL_XY_I  VectorParams1D=off  ShowAdditionalParam=off  OutDataTypeStr=double
  POSCONTROL_VEL_XY_IMAX1 : DataStoreMemory  DataStoreName=POSCONTROL_VEL_XY_IMAX  ReadBeforeWriteMsg=warning  WriteAfterWriteMsg=warning  WriteAfterReadMsg=warning  InitialValue=POSCONTROL_VEL_XY_IMAX  VectorParams1D=off  ShowAdditionalParam=off  OutDataTypeStr=double
  POSCONTROL_VEL_XY_I_inint1 : DataStoreMemory  DataStoreName=POSCONTROL_VEL_XY_I_inint  ReadBeforeWriteMsg=warning  WriteAfterWriteMsg=warning  WriteAfterReadMsg=warning  InitialValue=POSCONTROL_VEL_XY_I_inint  VectorParams1D=off  ShowAdditionalParam=off  OutDataTypeStr=double
  POSCONTROL_VEL_XY_P1 : DataStoreMemory  DataStoreName=POSCONTROL_VEL_XY_P  ReadBeforeWriteMsg=warning  WriteAfterWriteMsg=warning  WriteAfterReadMsg=warning  InitialValue=POSCONTROL_VEL_XY_P  VectorParams1D=off  ShowAdditionalParam=off  OutDataTypeStr=double
  POSCONTROL_VEL_Z_P1 : DataStoreMemory  DataStoreName=POSCONTROL_VEL_Z_P  ReadBeforeWriteMsg=warning  WriteAfterWriteMsg=warning  WriteAfterReadMsg=warning  InitialValue=POSCONTROL_VEL_Z_P  VectorParams1D=off  ShowAdditionalParam=off  OutDataTypeStr=double
  PathModeOut1 : DataStoreMemory  DataStoreName=PathModeOut_sl  ReadBeforeWriteMsg=warning  WriteAfterWriteMsg=warning  WriteAfterReadMsg=warning  InitialValue=PathModeOut_sl  VectorParams1D=off  ShowAdditionalParam=off  OutDataTypeStr=Bus: BUS_TASK_PATH_OutParam
  SKE_dem1 : DataStoreMemory  DataStoreName=SKE_dem  ReadBeforeWriteMsg=warning  WriteAfterWriteMsg=warning  WriteAfterReadMsg=warning  InitialValue=SKE_dem  VectorParams1D=off  ShowAdditionalParam=off  OutDataTypeStr=double
  SKE_est1 : DataStoreMemory  DataStoreName=SKE_est  ReadBeforeWriteMsg=warning  WriteAfterWriteMsg=warning  WriteAfterReadMsg=warning  InitialValue=SKE_est  VectorParams1D=off  ShowAdditionalParam=off  OutDataTypeStr=double
  SKEdot1 : DataStoreMemory  DataStoreName=SKEdot  ReadBeforeWriteMsg=warning  WriteAfterWriteMsg=warning  WriteAfterReadMsg=warning  InitialValue=SKEdot  VectorParams1D=off  ShowAdditionalParam=off  OutDataTypeStr=double
  SKEdot_dem1 : DataStoreMemory  DataStoreName=SKEdot_dem  ReadBeforeWriteMsg=warning  WriteAfterWriteMsg=warning  WriteAfterReadMsg=warning  InitialValue=SKEdot_dem  VectorParams1D=off  ShowAdditionalParam=off  OutDataTypeStr=double
  SPE_dem1 : DataStoreMemory  DataStoreName=SPE_dem  ReadBeforeWriteMsg=warning  WriteAfterWriteMsg=warning  WriteAfterReadMsg=warning  InitialValue=SPE_dem  VectorParams1D=off  ShowAdditionalParam=off  OutDataTypeStr=double
  SPE_est1 : DataStoreMemory  DataStoreName=SPE_est  ReadBeforeWriteMsg=warning  WriteAfterWriteMsg=warning  WriteAfterReadMsg=warning  InitialValue=SPE_est  VectorParams1D=off  ShowAdditionalParam=off  OutDataTypeStr=double
  SPEdot1 : DataStoreMemory  DataStoreName=SPEdot  ReadBeforeWriteMsg=warning  WriteAfterWriteMsg=warning  WriteAfterReadMsg=warning  InitialValue=SPEdot  VectorParams1D=off  ShowAdditionalParam=off  OutDataTypeStr=double
  SPEdot_dem1 : DataStoreMemory  DataStoreName=SPEdot_dem  ReadBeforeWriteMsg=warning  WriteAfterWriteMsg=warning  WriteAfterReadMsg=warning  InitialValue=SPEdot_dem  VectorParams1D=off  ShowAdditionalParam=off  OutDataTypeStr=double
  STE_error1 : DataStoreMemory  DataStoreName=STE_error  ReadBeforeWriteMsg=warning  WriteAfterWriteMsg=warning  WriteAfterReadMsg=warning  InitialValue=STE_error  VectorParams1D=off  ShowAdditionalParam=off  OutDataTypeStr=double
  STEdotErrLast1 : DataStoreMemory  DataStoreName=STEdotErrLast  ReadBeforeWriteMsg=warning  WriteAfterWriteMsg=warning  WriteAfterReadMsg=warning  InitialValue=STEdotErrLast  VectorParams1D=off  ShowAdditionalParam=off  OutDataTypeStr=double
  STEdot_max1 : DataStoreMemory  DataStoreName=STEdot_max  ReadBeforeWriteMsg=warning  WriteAfterWriteMsg=warning  WriteAfterReadMsg=warning  InitialValue=STEdot_max  VectorParams1D=off  ShowAdditionalParam=off  OutDataTypeStr=double
  STEdot_min1 : DataStoreMemory  DataStoreName=STEdot_min  ReadBeforeWriteMsg=warning  WriteAfterWriteMsg=warning  WriteAfterReadMsg=warning  InitialValue=STEdot_min  VectorParams1D=off  ShowAdditionalParam=off  OutDataTypeStr=double
  Scope{1..7,15,17,19..23,54,58,60,65..68,71..72,80..81,85..86,92..93,96..98,102,110,113,115,118..120,123,125..137,139..142,144..147,149,152..153,159..162,164..166,168..169,171..175,177..179} (81 alike) : Scope
  Scope{9..10,95,150..151,154,157..158} (8 alike) : Scope  NumInputPorts=3
  Scope{11..14,16,18,73,78,87..88,99..100,114,116..117,121..122,124,138,148,163,167,170,176} (24 alike) : Scope  NumInputPorts=2
  Scope{8,83,143,155} (4 alike) : Scope  NumInputPorts=4
  Sine Wave1 : Sin  Amplitude=50/57.3  Frequency=0.1*2*pi  SampleTime=0
  Sqrt : Sqrt  SaturateOnIntegerOverflow=on
  Subsystem : Subsystem
  Sum1 : Sum
  TAS_dem1 : DataStoreMemory  DataStoreName=TAS_dem  ReadBeforeWriteMsg=warning  WriteAfterWriteMsg=warning  WriteAfterReadMsg=warning  InitialValue=TAS_dem  VectorParams1D=off  ShowAdditionalParam=off  OutDataTypeStr=double
  TAS_dem_adj1 : DataStoreMemory  DataStoreName=TAS_dem_adj  ReadBeforeWriteMsg=warning  WriteAfterWriteMsg=warning  WriteAfterReadMsg=warning  InitialValue=TAS_dem_adj  VectorParams1D=off  ShowAdditionalParam=off  OutDataTypeStr=double
  TAS_rate_dem1 : DataStoreMemory  DataStoreName=TAS_rate_dem  ReadBeforeWriteMsg=warning  WriteAfterWriteMsg=warning  WriteAfterReadMsg=warning  InitialValue=TAS_rate_dem  VectorParams1D=off  ShowAdditionalParam=off  OutDataTypeStr=double
  TAS_state1 : DataStoreMemory  DataStoreName=TAS_state  ReadBeforeWriteMsg=warning  WriteAfterWriteMsg=warning  WriteAfterReadMsg=warning  InitialValue=TAS_state  VectorParams1D=off  ShowAdditionalParam=off  OutDataTypeStr=double
  TASmax1 : DataStoreMemory  DataStoreName=TASmax  ReadBeforeWriteMsg=warning  WriteAfterWriteMsg=warning  WriteAfterReadMsg=warning  InitialValue=TASmax  VectorParams1D=off  ShowAdditionalParam=off  OutDataTypeStr=double
  TASmin1 : DataStoreMemory  DataStoreName=TASmin  ReadBeforeWriteMsg=warning  WriteAfterWriteMsg=warning  WriteAfterReadMsg=warning  InitialValue=TASmin  VectorParams1D=off  ShowAdditionalParam=off  OutDataTypeStr=double
  THRmaxf1 : DataStoreMemory  DataStoreName=THRmaxf  ReadBeforeWriteMsg=warning  WriteAfterWriteMsg=warning  WriteAfterReadMsg=warning  InitialValue=THRmaxf  VectorParams1D=off  ShowAdditionalParam=off  OutDataTypeStr=double
  THRminf1 : DataStoreMemory  DataStoreName=THRminf  ReadBeforeWriteMsg=warning  WriteAfterWriteMsg=warning  WriteAfterReadMsg=warning  InitialValue=THRminf  VectorParams1D=off  ShowAdditionalParam=off  OutDataTypeStr=double
  Terminator{,1..2,6..11} (9 alike) : Terminator
  To Workspace2 : ToWorkspace  VariableName=current_loc_out1  SampleTime=-1
      settings: Save2DSignal=2-D array (concatenate along first dimension)
  To Workspace3 : ToWorkspace  VariableName=Xe_out1  SampleTime=-1
      settings: Save2DSignal=2-D array (concatenate along first dimension)
  Transpose : Math  Operator=transpose  SignedPower=on  SaturateOnIntegerOverflow=on
  Vz1 : DataStoreMemory  DataStoreName=Vz  ReadBeforeWriteMsg=warning  WriteAfterWriteMsg=warning  WriteAfterReadMsg=warning  InitialValue=Vz  ShowAdditionalParam=off  OutDataTypeStr=double
  WPcircle1 : DataStoreMemory  DataStoreName=WPcircle  ReadBeforeWriteMsg=warning  WriteAfterWriteMsg=warning  WriteAfterReadMsg=warning  InitialValue=WPcircle  VectorParams1D=off  ShowAdditionalParam=off  OutDataTypeStr=double
  accel_desired1 : DataStoreMemory  DataStoreName=accel_desired  ReadBeforeWriteMsg=warning  WriteAfterWriteMsg=warning  WriteAfterReadMsg=warning  InitialValue=accel_desired  VectorParams1D=off  ShowAdditionalParam=off  OutDataTypeStr=double
  accel_error1 : DataStoreMemory  DataStoreName=accel_error  ReadBeforeWriteMsg=warning  WriteAfterWriteMsg=warning  WriteAfterReadMsg=warning  InitialValue=accel_error  VectorParams1D=off  ShowAdditionalParam=off  OutDataTypeStr=double
  accel_last_z_cms1 : DataStoreMemory  DataStoreName=accel_last_z_cms  ReadBeforeWriteMsg=warning  WriteAfterWriteMsg=warning  WriteAfterReadMsg=warning  InitialValue=accel_last_z_cms  VectorParams1D=off  ShowAdditionalParam=off  OutDataTypeStr=double
  accel_pitch_max1 : DataStoreMemory  DataStoreName=accel_pitch_max  ReadBeforeWriteMsg=warning  WriteAfterWriteMsg=warning  WriteAfterReadMsg=warning  InitialValue=accel_pitch_max  VectorParams1D=off  ShowAdditionalParam=off  OutDataTypeStr=double
  accel_roll_max1 : DataStoreMemory  DataStoreName=accel_roll_max  ReadBeforeWriteMsg=warning  WriteAfterWriteMsg=warning  WriteAfterReadMsg=warning  InitialValue=accel_roll_max  VectorParams1D=off  ShowAdditionalParam=off  OutDataTypeStr=double
  accel_target1 : DataStoreMemory  DataStoreName=accel_target  ReadBeforeWriteMsg=warning  WriteAfterWriteMsg=warning  WriteAfterReadMsg=warning  InitialValue=accel_target  VectorParams1D=off  ShowAdditionalParam=off  OutDataTypeStr=double
  accel_x1 : DataStoreMemory  DataStoreName=accel_x  ReadBeforeWriteMsg=warning  WriteAfterWriteMsg=warning  WriteAfterReadMsg=warning  InitialValue=accel_x  ShowAdditionalParam=off  OutDataTypeStr=double
  accel_xy_angle_max1 : DataStoreMemory  DataStoreName=accel_xy_angle_max  ReadBeforeWriteMsg=warning  WriteAfterWriteMsg=warning  WriteAfterReadMsg=warning  InitialValue=accel_xy_angle_max  VectorParams1D=off  ShowAdditionalParam=off  OutDataTypeStr=double
  accel_xy_input1 : DataStoreMemory  DataStoreName=accel_xy_input  ReadBeforeWriteMsg=warning  WriteAfterWriteMsg=warning  WriteAfterReadMsg=warning  InitialValue=accel_xy_input  VectorParams1D=off  ShowAdditionalParam=off  OutDataTypeStr=double
  accel_y1 : DataStoreMemory  DataStoreName=accel_y  ReadBeforeWriteMsg=warning  WriteAfterWriteMsg=warning  WriteAfterReadMsg=warning  InitialValue=accel_y  ShowAdditionalParam=off  OutDataTypeStr=double
  accel_yaw_max1 : DataStoreMemory  DataStoreName=accel_yaw_max  ReadBeforeWriteMsg=warning  WriteAfterWriteMsg=warning  WriteAfterReadMsg=warning  InitialValue=accel_yaw_max  VectorParams1D=off  ShowAdditionalParam=off  OutDataTypeStr=double
  accel_z1 : DataStoreMemory  DataStoreName=accel_z  ReadBeforeWriteMsg=warning  WriteAfterWriteMsg=warning  WriteAfterReadMsg=warning  InitialValue=accel_z  ShowAdditionalParam=off  OutDataTypeStr=double
  aerodynamic_load_factor1 : DataStoreMemory  DataStoreName=aerodynamic_load_factor  ReadBeforeWriteMsg=warning  WriteAfterWriteMsg=warning  WriteAfterReadMsg=warning  InitialValue=aerodynamic_load_factor  ShowAdditionalParam=off  OutDataTypeStr=double
  air_density_ratio1 : DataStoreMemory  DataStoreName=air_density_ratio  ReadBeforeWriteMsg=warning  WriteAfterWriteMsg=warning  WriteAfterReadMsg=warning  InitialValue=air_density_ratio  VectorParams1D=off  ShowAdditionalParam=off  OutDataTypeStr=double
  airspeed_max1 : DataStoreMemory  DataStoreName=airspeed_max  ReadBeforeWriteMsg=warning  WriteAfterWriteMsg=warning  WriteAfterReadMsg=warning  InitialValue=airspeed_max  VectorParams1D=off  ShowAdditionalParam=off  OutDataTypeStr=double
  airspeed_min1 : DataStoreMemory  DataStoreName=airspeed_min  ReadBeforeWriteMsg=warning  WriteAfterWriteMsg=warning  WriteAfterReadMsg=warning  InitialValue=airspeed_min  VectorParams1D=off  ShowAdditionalParam=off  OutDataTypeStr=double
  algo_dbg_param : DataStoreMemory  DataStoreName=algo_dbg_param  ReadBeforeWriteMsg=warning  WriteAfterWriteMsg=warning  WriteAfterReadMsg=warning  InitialValue=algo_dbg_param  VectorParams1D=off  ShowAdditionalParam=off  OutDataTypeStr=Bus: BUS_CTRL_dbg_param
  algo_remote_ct_st : DataStoreMemory  DataStoreName=algo_remote_ct_st  ReadBeforeWriteMsg=warning  WriteAfterWriteMsg=warning  WriteAfterReadMsg=warning  InitialValue=algo_remote_ct_st  VectorParams1D=off  ShowAdditionalParam=off  OutDataTypeStr=Bus:BUS_CTRL_remote_ct_st
  althold_lean_angle_max1 : DataStoreMemory  DataStoreName=althold_lean_angle_max  ReadBeforeWriteMsg=warning  WriteAfterWriteMsg=warning  WriteAfterReadMsg=warning  InitialValue=althold_lean_angle_max  VectorParams1D=off  ShowAdditionalParam=off  OutDataTypeStr=double
  ang_vel_pitch_max1 : DataStoreMemory  DataStoreName=ang_vel_pitch_max  ReadBeforeWriteMsg=warning  WriteAfterWriteMsg=warning  WriteAfterReadMsg=warning  InitialValue=ang_vel_pitch_max  ShowAdditionalParam=off  OutDataTypeStr=double
  ang_vel_roll_max1 : DataStoreMemory  DataStoreName=ang_vel_roll_max  ReadBeforeWriteMsg=warning  WriteAfterWriteMsg=warning  WriteAfterReadMsg=warning  InitialValue=ang_vel_roll_max  ShowAdditionalParam=off  OutDataTypeStr=double
  ang_vel_yaw_max1 : DataStoreMemory  DataStoreName=ang_vel_yaw_max  ReadBeforeWriteMsg=warning  WriteAfterWriteMsg=warning  WriteAfterReadMsg=warning  InitialValue=ang_vel_yaw_max  ShowAdditionalParam=off  OutDataTypeStr=double
  angle_boost1 : DataStoreMemory  DataStoreName=angle_boost  ReadBeforeWriteMsg=warning  WriteAfterWriteMsg=warning  WriteAfterReadMsg=warning  InitialValue=angle_boost  VectorParams1D=off  ShowAdditionalParam=off  OutDataTypeStr=double
  angle_boost_enabled1 : DataStoreMemory  DataStoreName=angle_boost_enabled  ReadBeforeWriteMsg=warning  WriteAfterWriteMsg=warning  WriteAfterReadMsg=warning  InitialValue=angle_boost_enabled  VectorParams1D=off  ShowAdditionalParam=off  OutDataTypeStr=double
  angle_limit_tc1 : DataStoreMemory  DataStoreName=angle_limit_tc  ReadBeforeWriteMsg=warning  WriteAfterWriteMsg=warning  WriteAfterReadMsg=warning  InitialValue=angle_limit_tc  VectorParams1D=off  ShowAdditionalParam=off  OutDataTypeStr=double
  armed1 : DataStoreMemory  DataStoreName=armed  ReadBeforeWriteMsg=warning  WriteAfterWriteMsg=warning  WriteAfterReadMsg=warning  InitialValue=armed  VectorParams1D=off  ShowAdditionalParam=off  OutDataTypeStr=double
  arspeed_filt1 : DataStoreMemory  DataStoreName=arspeed_filt  ReadBeforeWriteMsg=warning  WriteAfterWriteMsg=warning  WriteAfterReadMsg=warning  InitialValue=arspeed_filt  VectorParams1D=off  ShowAdditionalParam=off  OutDataTypeStr=double
  arspeed_temp1 : DataStoreMemory  DataStoreName=arspeed_temp  ReadBeforeWriteMsg=warning  WriteAfterWriteMsg=warning  WriteAfterReadMsg=warning  InitialValue=arspeed_temp  VectorParams1D=off  ShowAdditionalParam=off  OutDataTypeStr=double
  aspeed1 : DataStoreMemory  DataStoreName=aspeed  ReadBeforeWriteMsg=warning  WriteAfterWriteMsg=warning  WriteAfterReadMsg=warning  InitialValue=aspeed  ShowAdditionalParam=off  OutDataTypeStr=double
  aspeed_c2p1 : DataStoreMemory  DataStoreName=aspeed_c2p  ReadBeforeWriteMsg=warning  WriteAfterWriteMsg=warning  WriteAfterReadMsg=warning  InitialValue=aspeed_c2p  VectorParams1D=off  ShowAdditionalParam=off  OutDataTypeStr=double
  aspeed_c2ps1 : DataStoreMemory  DataStoreName=aspeed_c2ps  ReadBeforeWriteMsg=warning  WriteAfterWriteMsg=warning  WriteAfterReadMsg=warning  InitialValue=aspeed_c2ps  VectorParams1D=off  ShowAdditionalParam=off  OutDataTypeStr=double
  aspeed_cp1 : DataStoreMemory  DataStoreName=aspeed_cp  ReadBeforeWriteMsg=warning  WriteAfterWriteMsg=warning  WriteAfterReadMsg=warning  InitialValue=aspeed_cp  VectorParams1D=off  ShowAdditionalParam=off  OutDataTypeStr=double
  attitude_ang_error1 : DataStoreMemory  DataStoreName=attitude_ang_error  ReadBeforeWriteMsg=warning  WriteAfterWriteMsg=warning  WriteAfterReadMsg=warning  InitialValue=attitude_ang_error  VectorParams1D=off  ShowAdditionalParam=off  OutDataTypeStr=double
  attitude_error_vector1 : DataStoreMemory  DataStoreName=attitude_error_vector  ReadBeforeWriteMsg=warning  WriteAfterWriteMsg=warning  WriteAfterReadMsg=warning  InitialValue=attitude_error_vector  VectorParams1D=off  ShowAdditionalParam=off  OutDataTypeStr=double
  attitude_target_ang_vel1 : DataStoreMemory  DataStoreName=attitude_target_ang_vel  ReadBeforeWriteMsg=warning  WriteAfterWriteMsg=warning  WriteAfterReadMsg=warning  InitialValue=attitude_target_ang_vel  VectorParams1D=off  ShowAdditionalParam=off  OutDataTypeStr=double
  attitude_target_euler_angle1 : DataStoreMemory  DataStoreName=attitude_target_euler_angle  ReadBeforeWriteMsg=warning  WriteAfterWriteMsg=warning  WriteAfterReadMsg=warning  InitialValue=attitude_target_euler_angle  VectorParams1D=off  ShowAdditionalParam=off  OutDataTypeStr=double
  attitude_target_euler_rate1 : DataStoreMemory  DataStoreName=attitude_target_euler_rate  ReadBeforeWriteMsg=warning  WriteAfterWriteMsg=warning  WriteAfterReadMsg=warning  InitialValue=attitude_target_euler_rate  VectorParams1D=off  ShowAdditionalParam=off  OutDataTypeStr=double
  attitude_target_quat1 : DataStoreMemory  DataStoreName=attitude_target_quat  ReadBeforeWriteMsg=warning  WriteAfterWriteMsg=warning  WriteAfterReadMsg=warning  InitialValue=attitude_target_quat  VectorParams1D=off  ShowAdditionalParam=off  OutDataTypeStr=double
  bearing_error1 : DataStoreMemory  DataStoreName=bearing_error  ReadBeforeWriteMsg=warning  WriteAfterWriteMsg=warning  WriteAfterReadMsg=warning  InitialValue=bearing_error  VectorParams1D=off  ShowAdditionalParam=off  OutDataTypeStr=double
  center_WP1 : DataStoreMemory  DataStoreName=center_WP  ReadBeforeWriteMsg=warning  WriteAfterWriteMsg=warning  WriteAfterReadMsg=warning  InitialValue=center_WP  VectorParams1D=off  ShowAdditionalParam=off  OutDataTypeStr=double
  climb_rate1 : DataStoreMemory  DataStoreName=climb_rate  ReadBeforeWriteMsg=warning  WriteAfterWriteMsg=warning  WriteAfterReadMsg=warning  InitialValue=climb_rate  VectorParams1D=off  ShowAdditionalParam=off  OutDataTypeStr=double
  climb_rate_cms1 : DataStoreMemory  DataStoreName=climb_rate_cms  ReadBeforeWriteMsg=warning  WriteAfterWriteMsg=warning  WriteAfterReadMsg=warning  InitialValue=climb_rate_cms  VectorParams1D=off  ShowAdditionalParam=off  OutDataTypeStr=double
  crosstrack_error1 : DataStoreMemory  DataStoreName=crosstrack_error  ReadBeforeWriteMsg=warning  WriteAfterWriteMsg=warning  WriteAfterReadMsg=warning  InitialValue=crosstrack_error  VectorParams1D=off  ShowAdditionalParam=off  OutDataTypeStr=double
  curr_alt1 : DataStoreMemory  DataStoreName=curr_alt  ReadBeforeWriteMsg=warning  WriteAfterWriteMsg=warning  WriteAfterReadMsg=warning  InitialValue=curr_alt  VectorParams1D=off  ShowAdditionalParam=off  OutDataTypeStr=double
  curr_pos1 : DataStoreMemory  DataStoreName=curr_pos  ReadBeforeWriteMsg=warning  WriteAfterWriteMsg=warning  WriteAfterReadMsg=warning  InitialValue=curr_pos  ShowAdditionalParam=off  OutDataTypeStr=double
  curr_vel1 : DataStoreMemory  DataStoreName=curr_vel  ReadBeforeWriteMsg=warning  WriteAfterWriteMsg=warning  WriteAfterReadMsg=warning  InitialValue=curr_vel  VectorParams1D=off  ShowAdditionalParam=off  OutDataTypeStr=double
  current_loc1 : DataStoreMemory  DataStoreName=current_loc  ReadBeforeWriteMsg=warning  WriteAfterWriteMsg=warning  WriteAfterReadMsg=warning  InitialValue=current_loc  VectorParams1D=off  ShowAdditionalParam=off  OutDataTypeStr=double
  current_tilt1 : DataStoreMemory  DataStoreName=current_tilt  ReadBeforeWriteMsg=warning  WriteAfterWriteMsg=warning  WriteAfterReadMsg=warning  InitialValue=current_tilt  VectorParams1D=off  ShowAdditionalParam=off  OutDataTypeStr=double
  data_is_stale1 : DataStoreMemory  DataStoreName=data_is_stale  ReadBeforeWriteMsg=warning  WriteAfterWriteMsg=warning  WriteAfterReadMsg=warning  InitialValue=data_is_stale  VectorParams1D=off  ShowAdditionalParam=off  OutDataTypeStr=double
  desired_rate_pitch1 : DataStoreMemory  DataStoreName=desired_rate_pitch  ReadBeforeWriteMsg=warning  WriteAfterWriteMsg=warning  WriteAfterReadMsg=warning  InitialValue=desired_rate_pitch  VectorParams1D=off  ShowAdditionalParam=off  OutDataTypeStr=double
  desired_rate_roll1 : DataStoreMemory  DataStoreName=desired_rate_roll  ReadBeforeWriteMsg=warning  WriteAfterWriteMsg=warning  WriteAfterReadMsg=warning  InitialValue=desired_rate_roll  VectorParams1D=off  ShowAdditionalParam=off  OutDataTypeStr=double
  disable_integrator_pitch1 : DataStoreMemory  DataStoreName=disable_integrator_pitch  ReadBeforeWriteMsg=warning  WriteAfterWriteMsg=warning  WriteAfterReadMsg=warning  InitialValue=disable_integrator_pitch  ShowAdditionalParam=off  OutDataTypeStr=double
  disable_integrator_roll1 : DataStoreMemory  DataStoreName=disable_integrator_roll  ReadBeforeWriteMsg=warning  WriteAfterWriteMsg=warning  WriteAfterReadMsg=warning  InitialValue=disable_integrator_roll  ShowAdditionalParam=off  OutDataTypeStr=double
  disable_integrator_yaw1 : DataStoreMemory  DataStoreName=disable_integrator_yaw  ReadBeforeWriteMsg=warning  WriteAfterWriteMsg=warning  WriteAfterReadMsg=warning  InitialValue=disable_integrator_yaw  ShowAdditionalParam=off  OutDataTypeStr=double
  dist_min1 : DataStoreMemory  DataStoreName=dist_min  ReadBeforeWriteMsg=warning  WriteAfterWriteMsg=warning  WriteAfterReadMsg=warning  InitialValue=dist_min  VectorParams1D=off  ShowAdditionalParam=off  OutDataTypeStr=double
  dt1 : DataStoreMemory  DataStoreName=dt  ReadBeforeWriteMsg=warning  WriteAfterWriteMsg=warning  WriteAfterReadMsg=warning  InitialValue=dt  ShowAdditionalParam=off  OutDataTypeStr=double
  ff_throttle : DataStoreMemory  DataStoreName=ff_throttle  ReadBeforeWriteMsg=warning  WriteAfterWriteMsg=warning  WriteAfterReadMsg=warning  InitialValue=ff_throttle  VectorParams1D=off  ShowAdditionalParam=off  OutDataTypeStr=double
  freeze_ff_z1 : DataStoreMemory  DataStoreName=freeze_ff_z  ReadBeforeWriteMsg=warning  WriteAfterWriteMsg=warning  WriteAfterReadMsg=warning  InitialValue=freeze_ff_z  VectorParams1D=off  ShowAdditionalParam=off  OutDataTypeStr=double
  gains_D_pitch1 : DataStoreMemory  DataStoreName=gains_D_pitch  ReadBeforeWriteMsg=warning  WriteAfterWriteMsg=warning  WriteAfterReadMsg=warning  InitialValue=gains_D_pitch  ShowAdditionalParam=off  OutDataTypeStr=double
  gains_D_pitch_inint : DataStoreMemory  DataStoreName=gains_D_pitch_inint  ReadBeforeWriteMsg=warning  WriteAfterWriteMsg=warning  WriteAfterReadMsg=warning  InitialValue=gains_D_pitch_inint  VectorParams1D=off  ShowAdditionalParam=off  OutDataTypeStr=double
  gains_D_roll1 : DataStoreMemory  DataStoreName=gains_D_roll  ReadBeforeWriteMsg=warning  WriteAfterWriteMsg=warning  WriteAfterReadMsg=warning  InitialValue=gains_D_roll  ShowAdditionalParam=off  OutDataTypeStr=double
  gains_D_roll_inint : DataStoreMemory  DataStoreName=gains_D_roll_inint  ReadBeforeWriteMsg=warning  WriteAfterWriteMsg=warning  WriteAfterReadMsg=warning  InitialValue=gains_D_roll_inint  VectorParams1D=off  ShowAdditionalParam=off  OutDataTypeStr=double
  gains_FF1 : DataStoreMemory  DataStoreName=gains_FF_pitch  ReadBeforeWriteMsg=warning  WriteAfterWriteMsg=warning  WriteAfterReadMsg=warning  InitialValue=gains_FF_pitch  ShowAdditionalParam=off  OutDataTypeStr=double
  gains_FF_roll1 : DataStoreMemory  DataStoreName=gains_FF_roll  ReadBeforeWriteMsg=warning  WriteAfterWriteMsg=warning  WriteAfterReadMsg=warning  InitialValue=gains_FF_roll  ShowAdditionalParam=off  OutDataTypeStr=double
  gains_I_pitch1 : DataStoreMemory  DataStoreName=gains_I_pitch  ReadBeforeWriteMsg=warning  WriteAfterWriteMsg=warning  WriteAfterReadMsg=warning  InitialValue=gains_I_pitch  ShowAdditionalParam=off  OutDataTypeStr=double
  gains_I_roll1 : DataStoreMemory  DataStoreName=gains_I_roll  ReadBeforeWriteMsg=warning  WriteAfterWriteMsg=warning  WriteAfterReadMsg=warning  InitialValue=gains_I_roll  ShowAdditionalParam=off  OutDataTypeStr=double
  gains_P1 : DataStoreMemory  DataStoreName=gains_P_pitch  ReadBeforeWriteMsg=warning  WriteAfterWriteMsg=warning  WriteAfterReadMsg=warning  InitialValue=gains_P_pitch  ShowAdditionalParam=off  OutDataTypeStr=double
  gains_P_roll1 : DataStoreMemory  DataStoreName=gains_P_roll  ReadBeforeWriteMsg=warning  WriteAfterWriteMsg=warning  WriteAfterReadMsg=warning  InitialValue=gains_P_roll  ShowAdditionalParam=off  OutDataTypeStr=double
  gains_imax_pitch1 : DataStoreMemory  DataStoreName=gains_imax_pitch  ReadBeforeWriteMsg=warning  WriteAfterWriteMsg=warning  WriteAfterReadMsg=warning  InitialValue=gains_imax_pitch  ShowAdditionalParam=off  OutDataTypeStr=double
  gains_imax_roll1 : DataStoreMemory  DataStoreName=gains_imax_roll  ReadBeforeWriteMsg=warning  WriteAfterWriteMsg=warning  WriteAfterReadMsg=warning  InitialValue=gains_imax_roll  ShowAdditionalParam=off  OutDataTypeStr=double
  gains_rmax1 : DataStoreMemory  DataStoreName=gains_rmax_roll  ReadBeforeWriteMsg=warning  WriteAfterWriteMsg=warning  WriteAfterReadMsg=warning  InitialValue=gains_rmax_roll  ShowAdditionalParam=off  OutDataTypeStr=double
  gains_rmax_pitch1 : DataStoreMemory  DataStoreName=gains_rmax_pitch  ReadBeforeWriteMsg=warning  WriteAfterWriteMsg=warning  WriteAfterReadMsg=warning  InitialValue=gains_rmax_pitch  ShowAdditionalParam=off  OutDataTypeStr=double
  gains_tau_pitch1 : DataStoreMemory  DataStoreName=gains_tau_pitch  ReadBeforeWriteMsg=warning  WriteAfterWriteMsg=warning  WriteAfterReadMsg=warning  InitialValue=gains_tau_pitch  ShowAdditionalParam=off  OutDataTypeStr=double
  gains_tau_roll1 : DataStoreMemory  DataStoreName=gains_tau_roll  ReadBeforeWriteMsg=warning  WriteAfterWriteMsg=warning  WriteAfterReadMsg=warning  InitialValue=gains_tau_roll  ShowAdditionalParam=off  OutDataTypeStr=double
  get_vector_xy_from_origin_NE1 : MATLAB Function  TreatAsAtomicUnit=on
  gn3 : Constant  Value=[0;0;GRAVITY_MSS]
  gn4 : Constant  Value=[0;0;GRAVITY_MSS]
  groundspeed_vector1 : DataStoreMemory  DataStoreName=groundspeed_vector  ReadBeforeWriteMsg=warning  WriteAfterWriteMsg=warning  WriteAfterReadMsg=warning  InitialValue=groundspeed_vector  VectorParams1D=off  ShowAdditionalParam=off  OutDataTypeStr=double
  gyro_x1 : DataStoreMemory  DataStoreName=gyro_x  ReadBeforeWriteMsg=warning  WriteAfterWriteMsg=warning  WriteAfterReadMsg=warning  InitialValue=gyro_x  ShowAdditionalParam=off  OutDataTypeStr=double
  gyro_y1 : DataStoreMemory  DataStoreName=gyro_y  ReadBeforeWriteMsg=warning  WriteAfterWriteMsg=warning  WriteAfterReadMsg=warning  InitialValue=gyro_y  ShowAdditionalParam=off  OutDataTypeStr=double
  gyro_z1 : DataStoreMemory  DataStoreName=gyro_z  ReadBeforeWriteMsg=warning  WriteAfterWriteMsg=warning  WriteAfterReadMsg=warning  InitialValue=gyro_z  ShowAdditionalParam=off  OutDataTypeStr=double
  heading_hold : DataStoreMemory  DataStoreName=heading_hold  ReadBeforeWriteMsg=warning  WriteAfterWriteMsg=warning  WriteAfterReadMsg=warning  InitialValue=heading_hold  VectorParams1D=off  ShowAdditionalParam=off  OutDataTypeStr=double
  height1 : DataStoreMemory  DataStoreName=height  ReadBeforeWriteMsg=warning  WriteAfterWriteMsg=warning  WriteAfterReadMsg=warning  InitialValue=height  VectorParams1D=off  ShowAdditionalParam=off  OutDataTypeStr=double
  hgt_dem1 : DataStoreMemory  DataStoreName=hgt_dem  ReadBeforeWriteMsg=warning  WriteAfterWriteMsg=warning  WriteAfterReadMsg=warning  InitialValue=hgt_dem  VectorParams1D=off  ShowAdditionalParam=off  OutDataTypeStr=double
  hgt_dem_adj1 : DataStoreMemory  DataStoreName=hgt_dem_adj  ReadBeforeWriteMsg=warning  WriteAfterWriteMsg=warning  WriteAfterReadMsg=warning  InitialValue=hgt_dem_adj  VectorParams1D=off  ShowAdditionalParam=off  OutDataTypeStr=double
  hgt_dem_adj_last1 : DataStoreMemory  DataStoreName=hgt_dem_adj_last  ReadBeforeWriteMsg=warning  WriteAfterWriteMsg=warning  WriteAfterReadMsg=warning  InitialValue=hgt_dem_adj_last  VectorParams1D=off  ShowAdditionalParam=off  OutDataTypeStr=double
  hgt_dem_cm1 : DataStoreMemory  DataStoreName=hgt_dem_cm  ReadBeforeWriteMsg=warning  WriteAfterWriteMsg=warning  WriteAfterReadMsg=warning  InitialValue=hgt_dem_cm  VectorParams1D=off  ShowAdditionalParam=off  OutDataTypeStr=double
  hgt_dem_in_old1 : DataStoreMemory  DataStoreName=hgt_dem_in_old  ReadBeforeWriteMsg=warning  WriteAfterWriteMsg=warning  WriteAfterReadMsg=warning  InitialValue=hgt_dem_in_old  VectorParams1D=off  ShowAdditionalParam=off  OutDataTypeStr=double
  hgt_dem_prev1 : DataStoreMemory  DataStoreName=hgt_dem_prev  ReadBeforeWriteMsg=warning  WriteAfterWriteMsg=warning  WriteAfterReadMsg=warning  InitialValue=hgt_dem_prev  VectorParams1D=off  ShowAdditionalParam=off  OutDataTypeStr=double
  hgt_rate_dem1 : DataStoreMemory  DataStoreName=hgt_rate_dem  ReadBeforeWriteMsg=warning  WriteAfterWriteMsg=warning  WriteAfterReadMsg=warning  InitialValue=hgt_rate_dem  VectorParams1D=off  ShowAdditionalParam=off  OutDataTypeStr=double
  highest_airspeed1 : DataStoreMemory  DataStoreName=highest_airspeed  ReadBeforeWriteMsg=warning  WriteAfterWriteMsg=warning  WriteAfterReadMsg=warning  InitialValue=highest_airspeed  ShowAdditionalParam=off  OutDataTypeStr=double
  imax_yaw1 : DataStoreMemory  DataStoreName=imax_yaw  ReadBeforeWriteMsg=warning  WriteAfterWriteMsg=warning  WriteAfterReadMsg=warning  InitialValue=imax_yaw  ShowAdditionalParam=off  OutDataTypeStr=double
  inint1 : DataStoreMemory  DataStoreName=inint  ReadBeforeWriteMsg=warning  WriteAfterWriteMsg=warning  WriteAfterReadMsg=warning  InitialValue=inint  VectorParams1D=off  ShowAdditionalParam=off  OutDataTypeStr=double
  inint_hgt1 : DataStoreMemory  DataStoreName=inint_hgt  ReadBeforeWriteMsg=warning  WriteAfterWriteMsg=warning  WriteAfterReadMsg=warning  InitialValue=inint_hgt  VectorParams1D=off  ShowAdditionalParam=off  OutDataTypeStr=double
  input_euler_angle_roll_pitch_euler_rate_yaw4 : MATLAB Function  TreatAsAtomicUnit=on
  input_tc1 : DataStoreMemory  DataStoreName=input_tc  ReadBeforeWriteMsg=warning  WriteAfterWriteMsg=warning  WriteAfterReadMsg=warning  InitialValue=input_tc  VectorParams1D=off  ShowAdditionalParam=off  OutDataTypeStr=double
  integDTAS_state1 : DataStoreMemory  DataStoreName=integDTAS_state  ReadBeforeWriteMsg=warning  WriteAfterWriteMsg=warning  WriteAfterReadMsg=warning  InitialValue=integDTAS_state  VectorParams1D=off  ShowAdditionalParam=off  OutDataTypeStr=double
  integGain1 : DataStoreMemory  DataStoreName=integGain  ReadBeforeWriteMsg=warning  WriteAfterWriteMsg=warning  WriteAfterReadMsg=warning  InitialValue=integGain  VectorParams1D=off  ShowAdditionalParam=off  OutDataTypeStr=double
  integSEB_state1 : DataStoreMemory  DataStoreName=integSEB_state  ReadBeforeWriteMsg=warning  WriteAfterWriteMsg=warning  WriteAfterReadMsg=warning  InitialValue=integSEB_state  VectorParams1D=off  ShowAdditionalParam=off  OutDataTypeStr=double
  integTHR_state1 : DataStoreMemory  DataStoreName=integTHR_state  ReadBeforeWriteMsg=warning  WriteAfterWriteMsg=warning  WriteAfterReadMsg=warning  InitialValue=integTHR_state  VectorParams1D=off  ShowAdditionalParam=off  OutDataTypeStr=double
  integrator_yaw1 : DataStoreMemory  DataStoreName=integrator_yaw  ReadBeforeWriteMsg=warning  WriteAfterWriteMsg=warning  WriteAfterReadMsg=warning  InitialValue=integrator_yaw  ShowAdditionalParam=off  OutDataTypeStr=double
  inverted_flight1 : DataStoreMemory  DataStoreName=inverted_flight  ReadBeforeWriteMsg=warning  WriteAfterWriteMsg=warning  WriteAfterReadMsg=warning  InitialValue=inverted_flight  ShowAdditionalParam=off  OutDataTypeStr=double
  is_active_xy1 : DataStoreMemory  DataStoreName=is_active_xy  ReadBeforeWriteMsg=warning  WriteAfterWriteMsg=warning  WriteAfterReadMsg=warning  InitialValue=is_active_xy  VectorParams1D=off  ShowAdditionalParam=off  OutDataTypeStr=double
  is_active_z1 : DataStoreMemory  DataStoreName=is_active_z  ReadBeforeWriteMsg=warning  WriteAfterWriteMsg=warning  WriteAfterReadMsg=warning  InitialValue=is_active_z  VectorParams1D=off  ShowAdditionalParam=off  OutDataTypeStr=double
  k_aileron1 : DataStoreMemory  DataStoreName=k_aileron  ReadBeforeWriteMsg=warning  WriteAfterWriteMsg=warning  WriteAfterReadMsg=warning  InitialValue=k_aileron  ShowAdditionalParam=off  OutDataTypeStr=double
  k_aileronL : DataStoreMemory  DataStoreName=k_aileronL  ReadBeforeWriteMsg=warning  WriteAfterWriteMsg=warning  WriteAfterReadMsg=warning  InitialValue=k_aileronL  ShowAdditionalParam=off  OutDataTypeStr=double
  k_aileronR : DataStoreMemory  DataStoreName=k_aileronR  ReadBeforeWriteMsg=warning  WriteAfterWriteMsg=warning  WriteAfterReadMsg=warning  InitialValue=k_aileronR  ShowAdditionalParam=off  OutDataTypeStr=double
  k_elevator1 : DataStoreMemory  DataStoreName=k_elevator  ReadBeforeWriteMsg=warning  WriteAfterWriteMsg=warning  WriteAfterReadMsg=warning  InitialValue=k_elevator  ShowAdditionalParam=off  OutDataTypeStr=double
  k_flap : DataStoreMemory  DataStoreName=k_flap  ReadBeforeWriteMsg=warning  WriteAfterWriteMsg=warning  WriteAfterReadMsg=warning  InitialValue=k_flap  VectorParams1D=off  ShowAdditionalParam=off  OutDataTypeStr=double
  k_flap_Land : DataStoreMemory  DataStoreName=k_flap_Land  ReadBeforeWriteMsg=warning  WriteAfterWriteMsg=warning  WriteAfterReadMsg=warning  InitialValue=k_flap_Land  VectorParams1D=off  ShowAdditionalParam=off  OutDataTypeStr=double
  k_flap_TakeOff : DataStoreMemory  DataStoreName=k_flap_TakeOff  ReadBeforeWriteMsg=warning  WriteAfterWriteMsg=warning  WriteAfterReadMsg=warning  InitialValue=k_flap_TakeOff  VectorParams1D=off  ShowAdditionalParam=off  OutDataTypeStr=double
  k_rudder1 : DataStoreMemory  DataStoreName=k_rudder  ReadBeforeWriteMsg=warning  WriteAfterWriteMsg=warning  WriteAfterReadMsg=warning  InitialValue=k_rudder  ShowAdditionalParam=off  OutDataTypeStr=double
  k_throttle1 : DataStoreMemory  DataStoreName=k_throttle  ReadBeforeWriteMsg=warning  WriteAfterWriteMsg=warning  WriteAfterReadMsg=warning  InitialValue=k_throttle  ShowAdditionalParam=off  OutDataTypeStr=double
  k_throttle_c2p : DataStoreMemory  DataStoreName=k_throttle_c2p  ReadBeforeWriteMsg=warning  WriteAfterWriteMsg=warning  WriteAfterReadMsg=warning  InitialValue=k_throttle_c2p  VectorParams1D=off  ShowAdditionalParam=off  OutDataTypeStr=double
  kff_rudder_mix1 : DataStoreMemory  DataStoreName=kff_rudder_mix  ReadBeforeWriteMsg=warning  WriteAfterWriteMsg=warning  WriteAfterReadMsg=warning  InitialValue=kff_rudder_mix  ShowAdditionalParam=off  OutDataTypeStr=double
  kff_throttle_to_pitch1 : DataStoreMemory  DataStoreName=kff_throttle_to_pitch  ReadBeforeWriteMsg=warning  WriteAfterWriteMsg=warning  WriteAfterReadMsg=warning  InitialValue=kff_throttle_to_pitch  ShowAdditionalParam=off  OutDataTypeStr=double
  last_Nu1 : DataStoreMemory  DataStoreName=last_Nu  ReadBeforeWriteMsg=warning  WriteAfterWriteMsg=warning  WriteAfterReadMsg=warning  InitialValue=last_Nu  VectorParams1D=off  ShowAdditionalParam=off  OutDataTypeStr=double
  last_out_pitch1 : DataStoreMemory  DataStoreName=last_out_pitch  ReadBeforeWriteMsg=warning  WriteAfterWriteMsg=warning  WriteAfterReadMsg=warning  InitialValue=last_out_pitch  ShowAdditionalParam=off  OutDataTypeStr=double
  last_out_roll1 : DataStoreMemory  DataStoreName=last_out_roll  ReadBeforeWriteMsg=warning  WriteAfterWriteMsg=warning  WriteAfterReadMsg=warning  InitialValue=last_out_roll  ShowAdditionalParam=off  OutDataTypeStr=double
  last_out_yaw1 : DataStoreMemory  DataStoreName=last_out_yaw  ReadBeforeWriteMsg=warning  WriteAfterWriteMsg=warning  WriteAfterReadMsg=warning  InitialValue=last_out_yaw  ShowAdditionalParam=off  OutDataTypeStr=double
  last_pitch_dem1 : DataStoreMemory  DataStoreName=last_pitch_dem  ReadBeforeWriteMsg=warning  WriteAfterWriteMsg=warning  WriteAfterReadMsg=warning  InitialValue=last_pitch_dem  VectorParams1D=off  ShowAdditionalParam=off  OutDataTypeStr=double
  last_rate_hp_in_yaw1 : DataStoreMemory  DataStoreName=last_rate_hp_in_yaw  ReadBeforeWriteMsg=warning  WriteAfterWriteMsg=warning  WriteAfterReadMsg=warning  InitialValue=last_rate_hp_in_yaw  ShowAdditionalParam=off  OutDataTypeStr=double
  last_rate_hp_out_yaw1 : DataStoreMemory  DataStoreName=last_rate_hp_out_yaw  ReadBeforeWriteMsg=warning  WriteAfterWriteMsg=warning  WriteAfterReadMsg=warning  InitialValue=last_rate_hp_out_yaw  ShowAdditionalParam=off  OutDataTypeStr=double
  last_throttle_dem1 : DataStoreMemory  DataStoreName=last_throttle_dem  ReadBeforeWriteMsg=warning  WriteAfterWriteMsg=warning  WriteAfterReadMsg=warning  InitialValue=last_throttle_dem  VectorParams1D=off  ShowAdditionalParam=off  OutDataTypeStr=double
  latAccDem1 : DataStoreMemory  DataStoreName=latAccDem  ReadBeforeWriteMsg=warning  WriteAfterWriteMsg=warning  WriteAfterReadMsg=warning  InitialValue=latAccDem  VectorParams1D=off  ShowAdditionalParam=off  OutDataTypeStr=double
  leash1 : DataStoreMemory  DataStoreName=leash  ReadBeforeWriteMsg=warning  WriteAfterWriteMsg=warning  WriteAfterReadMsg=warning  InitialValue=POSCONTROL_LEASH_LENGTH_MIN  ShowAdditionalParam=off  OutDataTypeStr=double
  leash_down_z1 : DataStoreMemory  DataStoreName=leash_down_z  ReadBeforeWriteMsg=warning  WriteAfterWriteMsg=warning  WriteAfterReadMsg=warning  InitialValue=POSCONTROL_LEASH_LENGTH_MIN  ShowAdditionalParam=off  OutDataTypeStr=double
  leash_up_z1 : DataStoreMemory  DataStoreName=leash_up_z  ReadBeforeWriteMsg=warning  WriteAfterWriteMsg=warning  WriteAfterReadMsg=warning  InitialValue=POSCONTROL_LEASH_LENGTH_MIN  ShowAdditionalParam=off  OutDataTypeStr=double
  limit_accel_xy1 : DataStoreMemory  DataStoreName=limit_accel_xy  ReadBeforeWriteMsg=warning  WriteAfterWriteMsg=warning  WriteAfterReadMsg=warning  InitialValue=limit_accel_xy  VectorParams1D=off  ShowAdditionalParam=off  OutDataTypeStr=double
  limit_pos_down1 : DataStoreMemory  DataStoreName=limit_pos_down  ReadBeforeWriteMsg=warning  WriteAfterWriteMsg=warning  WriteAfterReadMsg=warning  InitialValue=limit_pos_down  VectorParams1D=off  ShowAdditionalParam=off  OutDataTypeStr=double
  limit_pos_up1 : DataStoreMemory  DataStoreName=limit_pos_up  ReadBeforeWriteMsg=warning  WriteAfterWriteMsg=warning  WriteAfterReadMsg=warning  InitialValue=limit_pos_up  VectorParams1D=off  ShowAdditionalParam=off  OutDataTypeStr=double
  limit_roll_pitch1 : DataStoreMemory  DataStoreName=limit_roll_pitch  ReadBeforeWriteMsg=warning  WriteAfterWriteMsg=warning  WriteAfterReadMsg=warning  InitialValue=limit_roll_pitch  VectorParams1D=off  ShowAdditionalParam=off  OutDataTypeStr=double
  limit_vel_down1 : DataStoreMemory  DataStoreName=limit_vel_down  ReadBeforeWriteMsg=warning  WriteAfterWriteMsg=warning  WriteAfterReadMsg=warning  InitialValue=limit_vel_down  VectorParams1D=off  ShowAdditionalParam=off  OutDataTypeStr=double
  limit_vel_up1 : DataStoreMemory  DataStoreName=limit_vel_up  ReadBeforeWriteMsg=warning  WriteAfterWriteMsg=warning  WriteAfterReadMsg=warning  InitialValue=limit_vel_up  ShowAdditionalParam=off  OutDataTypeStr=double
  limit_yaw1 : DataStoreMemory  DataStoreName=limit_yaw  ReadBeforeWriteMsg=warning  WriteAfterWriteMsg=warning  WriteAfterReadMsg=warning  InitialValue=limit_yaw  VectorParams1D=off  ShowAdditionalParam=off  OutDataTypeStr=double
  loc1 : DataStoreMemory  DataStoreName=loc  ReadBeforeWriteMsg=warning  WriteAfterWriteMsg=warning  WriteAfterReadMsg=warning  InitialValue=loc  VectorParams1D=off  ShowAdditionalParam=off  OutDataTypeStr=Bus: BUS_CTRL_wp
  loc_origin1 : DataStoreMemory  DataStoreName=loc_origin  ReadBeforeWriteMsg=warning  WriteAfterWriteMsg=warning  WriteAfterReadMsg=warning  InitialValue=loc_origin  VectorParams1D=off  ShowAdditionalParam=off  OutDataTypeStr=double
  loiter_bank_limit1 : DataStoreMemory  DataStoreName=loiter_bank_limit  ReadBeforeWriteMsg=warning  WriteAfterWriteMsg=warning  WriteAfterReadMsg=warning  InitialValue=loiter_bank_limit  VectorParams1D=off  ShowAdditionalParam=off  OutDataTypeStr=double
  loiter_direction1 : DataStoreMemory  DataStoreName=loiter_direction  ReadBeforeWriteMsg=warning  WriteAfterWriteMsg=warning  WriteAfterReadMsg=warning  InitialValue=loiter_direction  VectorParams1D=off  ShowAdditionalParam=off  OutDataTypeStr=double
  maxClimbRate1 : DataStoreMemory  DataStoreName=maxClimbRate  ReadBeforeWriteMsg=warning  WriteAfterWriteMsg=warning  WriteAfterReadMsg=warning  InitialValue=maxClimbRate  VectorParams1D=off  ShowAdditionalParam=off  OutDataTypeStr=double
  maxSinkRate1 : DataStoreMemory  DataStoreName=maxSinkRate  ReadBeforeWriteMsg=warning  WriteAfterWriteMsg=warning  WriteAfterReadMsg=warning  InitialValue=maxSinkRate  VectorParams1D=off  ShowAdditionalParam=off  OutDataTypeStr=double
  max_rate_neg1 : DataStoreMemory  DataStoreName=max_rate_neg  ReadBeforeWriteMsg=warning  WriteAfterWriteMsg=warning  WriteAfterReadMsg=warning  InitialValue=max_rate_neg  ShowAdditionalParam=off  OutDataTypeStr=double
  minSinkRate1 : DataStoreMemory  DataStoreName=minSinkRate  ReadBeforeWriteMsg=warning  WriteAfterWriteMsg=warning  WriteAfterReadMsg=warning  InitialValue=minSinkRate  VectorParams1D=off  ShowAdditionalParam=off  OutDataTypeStr=double
  mode1 : DataStoreMemory  DataStoreName=mode  ReadBeforeWriteMsg=warning  WriteAfterWriteMsg=warning  WriteAfterReadMsg=warning  InitialValue=mode  VectorParams1D=off  ShowAdditionalParam=off  OutDataTypeStr=double
  mode_L2 : DataStoreMemory  DataStoreName=mode_L1  ReadBeforeWriteMsg=warning  WriteAfterWriteMsg=warning  WriteAfterReadMsg=warning  InitialValue=mode_L1  VectorParams1D=off  ShowAdditionalParam=off  OutDataTypeStr=double
  motors_limit_roll_pitch1 : DataStoreMemory  DataStoreName=motors_limit_roll_pitch  ReadBeforeWriteMsg=warning  WriteAfterWriteMsg=warning  WriteAfterReadMsg=warning  InitialValue=motors_limit_roll_pitch  VectorParams1D=off  ShowAdditionalParam=off  OutDataTypeStr=double
  motors_limit_throttle_upper1 : DataStoreMemory  DataStoreName=motors_limit_throttle_upper  ReadBeforeWriteMsg=warning  WriteAfterWriteMsg=warning  WriteAfterReadMsg=warning  InitialValue=motors_limit_throttle_upper  VectorParams1D=off  ShowAdditionalParam=off  OutDataTypeStr=double
  motors_limit_yaw1 : DataStoreMemory  DataStoreName=motors_limit_yaw  ReadBeforeWriteMsg=warning  WriteAfterWriteMsg=warning  WriteAfterReadMsg=warning  InitialValue=motors_limit_yaw  VectorParams1D=off  ShowAdditionalParam=off  OutDataTypeStr=double
  nav_bearing1 : DataStoreMemory  DataStoreName=nav_bearing  ReadBeforeWriteMsg=warning  WriteAfterWriteMsg=warning  WriteAfterReadMsg=warning  InitialValue=nav_bearing  VectorParams1D=off  ShowAdditionalParam=off  OutDataTypeStr=double
  nav_pitch_cd1 : DataStoreMemory  DataStoreName=nav_pitch_cd  ReadBeforeWriteMsg=warning  WriteAfterWriteMsg=warning  WriteAfterReadMsg=warning  InitialValue=nav_pitch_cd  ShowAdditionalParam=off  OutDataTypeStr=double
  nav_roll_cd1 : DataStoreMemory  DataStoreName=nav_roll_cd  ReadBeforeWriteMsg=warning  WriteAfterWriteMsg=warning  WriteAfterReadMsg=warning  InitialValue=nav_roll_cd  ShowAdditionalParam=off  OutDataTypeStr=double
  next_WP1 : DataStoreMemory  DataStoreName=next_WP  ReadBeforeWriteMsg=warning  WriteAfterWriteMsg=warning  WriteAfterReadMsg=warning  InitialValue=next_WP  VectorParams1D=off  ShowAdditionalParam=off  OutDataTypeStr=double
  p_angle_pitch1 : DataStoreMemory  DataStoreName=p_angle_pitch  ReadBeforeWriteMsg=warning  WriteAfterWriteMsg=warning  WriteAfterReadMsg=warning  InitialValue=p_angle_pitch  VectorParams1D=off  ShowAdditionalParam=off  OutDataTypeStr=double
  p_angle_roll1 : DataStoreMemory  DataStoreName=p_angle_roll  ReadBeforeWriteMsg=warning  WriteAfterWriteMsg=warning  WriteAfterReadMsg=warning  InitialValue=p_angle_roll  ShowAdditionalParam=off  OutDataTypeStr=double
  p_angle_yaw1 : DataStoreMemory  DataStoreName=p_angle_yaw  ReadBeforeWriteMsg=warning  WriteAfterWriteMsg=warning  WriteAfterReadMsg=warning  InitialValue=p_angle_yaw  ShowAdditionalParam=off  OutDataTypeStr=double
  p_ff_throttle1 : DataStoreMemory  DataStoreName=p_ff_throttle  ReadBeforeWriteMsg=warning  WriteAfterWriteMsg=warning  WriteAfterReadMsg=warning  InitialValue=p_ff_throttle  VectorParams1D=off  ShowAdditionalParam=off  OutDataTypeStr=double
  p_k_elevator_c2p : DataStoreMemory  DataStoreName=p_k_elevator_c2p  ReadBeforeWriteMsg=warning  WriteAfterWriteMsg=warning  WriteAfterReadMsg=warning  InitialValue=p_k_elevator_c2p  VectorParams1D=off  ShowAdditionalParam=off  OutDataTypeStr=double
  p_plane_c2p1 : DataStoreMemory  DataStoreName=p_plane_c2p  ReadBeforeWriteMsg=warning  WriteAfterWriteMsg=warning  WriteAfterReadMsg=warning  InitialValue=p_plane_c2p  VectorParams1D=off  ShowAdditionalParam=off  OutDataTypeStr=double
  p_plane_cp1 : DataStoreMemory  DataStoreName=p_plane_cp  ReadBeforeWriteMsg=warning  WriteAfterWriteMsg=warning  WriteAfterReadMsg=warning  InitialValue=p_plane_cp  VectorParams1D=off  ShowAdditionalParam=off  OutDataTypeStr=double
  p_plane_p2c : DataStoreMemory  DataStoreName=p_plane_p2c  ReadBeforeWriteMsg=warning  WriteAfterWriteMsg=warning  WriteAfterReadMsg=warning  InitialValue=p_plane_p2c  VectorParams1D=off  ShowAdditionalParam=off  OutDataTypeStr=double
  p_tail_tilt1 : DataStoreMemory  DataStoreName=p_tail_tilt  ReadBeforeWriteMsg=warning  WriteAfterWriteMsg=warning  WriteAfterReadMsg=warning  InitialValue=p_tail_tilt  VectorParams1D=off  ShowAdditionalParam=off  OutDataTypeStr=double
  p_tilt_pitch_target1 : DataStoreMemory  DataStoreName=p_tilt_pitch_target  ReadBeforeWriteMsg=warning  WriteAfterWriteMsg=warning  WriteAfterReadMsg=warning  InitialValue=p_tilt_pitch_target  VectorParams1D=off  ShowAdditionalParam=off  OutDataTypeStr=double
  pid_accel_z_derivative1 : DataStoreMemory  DataStoreName=pid_accel_z_derivative  ReadBeforeWriteMsg=warning  WriteAfterWriteMsg=warning  WriteAfterReadMsg=warning  InitialValue=pid_accel_z_derivative  VectorParams1D=off  ShowAdditionalParam=off  OutDataTypeStr=double
  pid_accel_z_input1 : DataStoreMemory  DataStoreName=pid_accel_z_input  ReadBeforeWriteMsg=warning  WriteAfterWriteMsg=warning  WriteAfterReadMsg=warning  InitialValue=pid_accel_z_input  VectorParams1D=off  ShowAdditionalParam=off  OutDataTypeStr=double
  pid_accel_z_integrator1 : DataStoreMemory  DataStoreName=pid_accel_z_integrator  ReadBeforeWriteMsg=warning  WriteAfterWriteMsg=warning  WriteAfterReadMsg=warning  InitialValue=pid_accel_z_integrator  VectorParams1D=off  ShowAdditionalParam=off  OutDataTypeStr=double
  pid_accel_z_reset_filter1 : DataStoreMemory  DataStoreName=pid_accel_z_reset_filter  ReadBeforeWriteMsg=warning  WriteAfterWriteMsg=warning  WriteAfterReadMsg=warning  InitialValue=pid_accel_z_reset_filter  VectorParams1D=off  ShowAdditionalParam=off  OutDataTypeStr=double
  pid_info_D_pitch1 : DataStoreMemory  DataStoreName=pid_info_D_pitch  ReadBeforeWriteMsg=warning  WriteAfterWriteMsg=warning  WriteAfterReadMsg=warning  InitialValue=pid_info_D_pitch  ShowAdditionalParam=off  OutDataTypeStr=double
  pid_info_D_roll1 : DataStoreMemory  DataStoreName=pid_info_D_roll  ReadBeforeWriteMsg=warning  WriteAfterWriteMsg=warning  WriteAfterReadMsg=warning  InitialValue=pid_info_D_roll  ShowAdditionalParam=off  OutDataTypeStr=double
  pid_info_D_yaw1 : DataStoreMemory  DataStoreName=pid_info_D_yaw  ReadBeforeWriteMsg=warning  WriteAfterWriteMsg=warning  WriteAfterReadMsg=warning  InitialValue=pid_info_D_yaw  ShowAdditionalParam=off  OutDataTypeStr=double
  pid_info_FF1 : DataStoreMemory  DataStoreName=pid_info_FF_pitch  ReadBeforeWriteMsg=warning  WriteAfterWriteMsg=warning  WriteAfterReadMsg=warning  InitialValue=pid_info_FF_pitch  ShowAdditionalParam=off  OutDataTypeStr=double
  pid_info_FF_roll1 : DataStoreMemory  DataStoreName=pid_info_FF_roll  ReadBeforeWriteMsg=warning  WriteAfterWriteMsg=warning  WriteAfterReadMsg=warning  InitialValue=pid_info_FF_roll  ShowAdditionalParam=off  OutDataTypeStr=double
  pid_info_I_pitch1 : DataStoreMemory  DataStoreName=pid_info_I_pitch  ReadBeforeWriteMsg=warning  WriteAfterWriteMsg=warning  WriteAfterReadMsg=warning  InitialValue=pid_info_I_pitch  ShowAdditionalParam=off  OutDataTypeStr=double
  pid_info_I_roll1 : DataStoreMemory  DataStoreName=pid_info_I_roll  ReadBeforeWriteMsg=warning  WriteAfterWriteMsg=warning  WriteAfterReadMsg=warning  InitialValue=pid_info_I_roll  ShowAdditionalParam=off  OutDataTypeStr=double
  pid_info_I_yaw1 : DataStoreMemory  DataStoreName=pid_info_I_yaw  ReadBeforeWriteMsg=warning  WriteAfterWriteMsg=warning  WriteAfterReadMsg=warning  InitialValue=pid_info_I_yaw  ShowAdditionalParam=off  OutDataTypeStr=double
  pid_info_P_pitch1 : DataStoreMemory  DataStoreName=pid_info_P_pitch  ReadBeforeWriteMsg=warning  WriteAfterWriteMsg=warning  WriteAfterReadMsg=warning  InitialValue=pid_info_P_pitch  ShowAdditionalParam=off  OutDataTypeStr=double
  pid_info_P_roll1 : DataStoreMemory  DataStoreName=pid_info_P_roll  ReadBeforeWriteMsg=warning  WriteAfterWriteMsg=warning  WriteAfterReadMsg=warning  InitialValue=pid_info_P_roll  ShowAdditionalParam=off  OutDataTypeStr=double
  pid_info_actua_pitchl1 : DataStoreMemory  DataStoreName=pid_info_actual_pitch  ReadBeforeWriteMsg=warning  WriteAfterWriteMsg=warning  WriteAfterReadMsg=warning  InitialValue=pid_info_actual_pitch  ShowAdditionalParam=off  OutDataTypeStr=double
  pid_info_actual_roll1 : DataStoreMemory  DataStoreName=pid_info_actual_roll  ReadBeforeWriteMsg=warning  WriteAfterWriteMsg=warning  WriteAfterReadMsg=warning  InitialValue=pid_info_actual_roll  ShowAdditionalParam=off  OutDataTypeStr=double
  pid_info_desired_pitch1 : DataStoreMemory  DataStoreName=pid_info_desired_pitch  ReadBeforeWriteMsg=warning  WriteAfterWriteMsg=warning  WriteAfterReadMsg=warning  InitialValue=pid_info_desired_pitch  ShowAdditionalParam=off  OutDataTypeStr=double
  pid_info_desired_roll1 : DataStoreMemory  DataStoreName=pid_info_desired_roll  ReadBeforeWriteMsg=warning  WriteAfterWriteMsg=warning  WriteAfterReadMsg=warning  InitialValue=pid_info_desired_roll  ShowAdditionalParam=off  OutDataTypeStr=double
  pid_vel_xy_derivative1 : DataStoreMemory  DataStoreName=pid_vel_xy_derivative  ReadBeforeWriteMsg=warning  WriteAfterWriteMsg=warning  WriteAfterReadMsg=warning  InitialValue=pid_vel_xy_derivative  VectorParams1D=off  ShowAdditionalParam=off  OutDataTypeStr=double
  pid_vel_xy_input1 : DataStoreMemory  DataStoreName=pid_vel_xy_input  ReadBeforeWriteMsg=warning  WriteAfterWriteMsg=warning  WriteAfterReadMsg=warning  InitialValue=pid_vel_xy_input  VectorParams1D=off  ShowAdditionalParam=off  OutDataTypeStr=double
  pid_vel_xy_integrator1 : DataStoreMemory  DataStoreName=pid_vel_xy_integrator  ReadBeforeWriteMsg=warning  WriteAfterWriteMsg=warning  WriteAfterReadMsg=warning  InitialValue=pid_vel_xy_integrator  VectorParams1D=off  ShowAdditionalParam=off  OutDataTypeStr=double
  pid_vel_xy_reset_filter1 : DataStoreMemory  DataStoreName=pid_vel_xy_reset_filter  ReadBeforeWriteMsg=warning  WriteAfterWriteMsg=warning  WriteAfterReadMsg=warning  InitialValue=pid_vel_xy_reset_filter  VectorParams1D=off  ShowAdditionalParam=off  OutDataTypeStr=double
  pitch1 : DataStoreMemory  DataStoreName=pitch  ReadBeforeWriteMsg=warning  WriteAfterWriteMsg=warning  WriteAfterReadMsg=warning  InitialValue=pitch  ShowAdditionalParam=off  OutDataTypeStr=double
  pitch_dem1 : DataStoreMemory  DataStoreName=pitch_dem  ReadBeforeWriteMsg=warning  WriteAfterWriteMsg=warning  WriteAfterReadMsg=warning  InitialValue=pitch_dem  VectorParams1D=off  ShowAdditionalParam=off  OutDataTypeStr=double
  pitch_dem_unc1 : DataStoreMemory  DataStoreName=pitch_dem_unc  ReadBeforeWriteMsg=warning  WriteAfterWriteMsg=warning  WriteAfterReadMsg=warning  InitialValue=pitch_dem_unc  VectorParams1D=off  ShowAdditionalParam=off  OutDataTypeStr=double
  pitch_factor1 : DataStoreMemory  DataStoreName=pitch_factor  ReadBeforeWriteMsg=warning  WriteAfterWriteMsg=warning  WriteAfterReadMsg=warning  InitialValue=pitch_factor  VectorParams1D=off  ShowAdditionalParam=off  OutDataTypeStr=double
  pitch_in1 : DataStoreMemory  DataStoreName=pitch_in  ReadBeforeWriteMsg=warning  WriteAfterWriteMsg=warning  WriteAfterReadMsg=warning  InitialValue=pitch_in  VectorParams1D=off  ShowAdditionalParam=off  OutDataTypeStr=double
  pitch_limit_max_cd1 : DataStoreMemory  DataStoreName=pitch_limit_max_cd  ReadBeforeWriteMsg=warning  WriteAfterWriteMsg=warning  WriteAfterReadMsg=warning  InitialValue=pitch_limit_max_cd  VectorParams1D=off  ShowAdditionalParam=off  OutDataTypeStr=double
  pitch_limit_min_cd1 : DataStoreMemory  DataStoreName=pitch_limit_min_cd  ReadBeforeWriteMsg=warning  WriteAfterWriteMsg=warning  WriteAfterReadMsg=warning  InitialValue=pitch_limit_min_cd  VectorParams1D=off  ShowAdditionalParam=off  OutDataTypeStr=double
  pitch_max1 : DataStoreMemory  DataStoreName=pitch_max  ReadBeforeWriteMsg=warning  WriteAfterWriteMsg=warning  WriteAfterReadMsg=warning  InitialValue=pitch_max  VectorParams1D=off  ShowAdditionalParam=off  OutDataTypeStr=double
  pitch_max_limit1 : DataStoreMemory  DataStoreName=pitch_max_limit  ReadBeforeWriteMsg=warning  WriteAfterWriteMsg=warning  WriteAfterReadMsg=warning  InitialValue=pitch_max_limit  VectorParams1D=off  ShowAdditionalParam=off  OutDataTypeStr=double
  pitch_min1 : DataStoreMemory  DataStoreName=pitch_min  ReadBeforeWriteMsg=warning  WriteAfterWriteMsg=warning  WriteAfterReadMsg=warning  InitialValue=pitch_min  VectorParams1D=off  ShowAdditionalParam=off  OutDataTypeStr=double
  pitch_target1 : DataStoreMemory  DataStoreName=pitch_target  ReadBeforeWriteMsg=warning  WriteAfterWriteMsg=warning  WriteAfterReadMsg=warning  InitialValue=pitch_target  VectorParams1D=off  ShowAdditionalParam=off  OutDataTypeStr=double
  pitch_target_c2p : DataStoreMemory  DataStoreName=pitch_target_c2p  ReadBeforeWriteMsg=warning  WriteAfterWriteMsg=warning  WriteAfterReadMsg=warning  InitialValue=pitch_target_c2p  VectorParams1D=off  ShowAdditionalParam=off  OutDataTypeStr=double
  pitch_target_p2c : DataStoreMemory  DataStoreName=pitch_target_p2c  ReadBeforeWriteMsg=warning  WriteAfterWriteMsg=warning  WriteAfterReadMsg=warning  InitialValue=pitch_target_p2c  VectorParams1D=off  ShowAdditionalParam=off  OutDataTypeStr=double
  pitch_target_pilot1 : DataStoreMemory  DataStoreName=pitch_target_pilot  ReadBeforeWriteMsg=warning  WriteAfterWriteMsg=warning  WriteAfterReadMsg=warning  InitialValue=pitch_target_pilot  VectorParams1D=off  ShowAdditionalParam=off  OutDataTypeStr=double
  plane_mode : DataStoreMemory  DataStoreName=plane_mode  ReadBeforeWriteMsg=warning  WriteAfterWriteMsg=warning  WriteAfterReadMsg=warning  InitialValue=plane_mode  VectorParams1D=off  ShowAdditionalParam=off  OutDataTypeStr=Enum: ENUM_plane_mode
  pos_error1 : DataStoreMemory  DataStoreName=pos_error  ReadBeforeWriteMsg=warning  WriteAfterWriteMsg=warning  WriteAfterReadMsg=warning  InitialValue=pos_error  VectorParams1D=off  ShowAdditionalParam=off  OutDataTypeStr=double
  pos_target1 : DataStoreMemory  DataStoreName=pos_target  ReadBeforeWriteMsg=warning  WriteAfterWriteMsg=warning  WriteAfterReadMsg=warning  InitialValue=pos_target  VectorParams1D=off  ShowAdditionalParam=off  OutDataTypeStr=double
  prev_WP1 : DataStoreMemory  DataStoreName=prev_WP  ReadBeforeWriteMsg=warning  WriteAfterWriteMsg=warning  WriteAfterReadMsg=warning  InitialValue=prev_WP  VectorParams1D=off  ShowAdditionalParam=off  OutDataTypeStr=double
  ptchDamp1 : DataStoreMemory  DataStoreName=ptchDamp  ReadBeforeWriteMsg=warning  WriteAfterWriteMsg=warning  WriteAfterReadMsg=warning  InitialValue=ptchDamp  VectorParams1D=off  ShowAdditionalParam=off  OutDataTypeStr=double
  pwm_max1 : DataStoreMemory  DataStoreName=pwm_max  ReadBeforeWriteMsg=warning  WriteAfterWriteMsg=warning  WriteAfterReadMsg=warning  InitialValue=pwm_max  ShowAdditionalParam=off  OutDataTypeStr=double
  pwm_min1 : DataStoreMemory  DataStoreName=pwm_min  ReadBeforeWriteMsg=warning  WriteAfterWriteMsg=warning  WriteAfterReadMsg=warning  InitialValue=pwm_min  ShowAdditionalParam=off  OutDataTypeStr=double
  pwm_out1 : DataStoreMemory  DataStoreName=pwm_out  ReadBeforeWriteMsg=warning  WriteAfterWriteMsg=warning  WriteAfterReadMsg=warning  InitialValue=pwm_out  ShowAdditionalParam=off  OutDataTypeStr=double
  pwm_tail : DataStoreMemory  DataStoreName=pwm_tail  ReadBeforeWriteMsg=warning  WriteAfterWriteMsg=warning  WriteAfterReadMsg=warning  InitialValue=pwm_tail  VectorParams1D=off  ShowAdditionalParam=off  OutDataTypeStr=double
  radius1 : DataStoreMemory  DataStoreName=radius  ReadBeforeWriteMsg=warning  WriteAfterWriteMsg=warning  WriteAfterReadMsg=warning  InitialValue=radius  VectorParams1D=off  ShowAdditionalParam=off  OutDataTypeStr=double
  rate_bf_ff_enabled1 : DataStoreMemory  DataStoreName=rate_bf_ff_enabled  ReadBeforeWriteMsg=warning  WriteAfterWriteMsg=warning  WriteAfterReadMsg=warning  InitialValue=rate_bf_ff_enabled  ShowAdditionalParam=off  OutDataTypeStr=double
  rate_pitch_pid_derivative1 : DataStoreMemory  DataStoreName=rate_pitch_pid_derivative  ReadBeforeWriteMsg=warning  WriteAfterWriteMsg=warning  WriteAfterReadMsg=warning  InitialValue=rate_pitch_pid_derivative  VectorParams1D=off  ShowAdditionalParam=off  OutDataTypeStr=double
  rate_pitch_pid_input1 : DataStoreMemory  DataStoreName=rate_pitch_pid_input  ReadBeforeWriteMsg=warning  WriteAfterWriteMsg=warning  WriteAfterReadMsg=warning  InitialValue=rate_pitch_pid_input  VectorParams1D=off  ShowAdditionalParam=off  OutDataTypeStr=double
  rate_pitch_pid_integrator1 : DataStoreMemory  DataStoreName=rate_pitch_pid_integrator  ReadBeforeWriteMsg=warning  WriteAfterWriteMsg=warning  WriteAfterReadMsg=warning  InitialValue=rate_pitch_pid_integrator  VectorParams1D=off  ShowAdditionalParam=off  OutDataTypeStr=double
  rate_pitch_pid_reset_filter1 : DataStoreMemory  DataStoreName=rate_pitch_pid_reset_filter  ReadBeforeWriteMsg=warning  WriteAfterWriteMsg=warning  WriteAfterReadMsg=warning  InitialValue=rate_pitch_pid_reset_filter  VectorParams1D=off  ShowAdditionalParam=off  OutDataTypeStr=double
  rate_roll_pid_derivative1 : DataStoreMemory  DataStoreName=rate_roll_pid_derivative  ReadBeforeWriteMsg=warning  WriteAfterWriteMsg=warning  WriteAfterReadMsg=warning  InitialValue=rate_roll_pid_derivative  VectorParams1D=off  ShowAdditionalParam=off  OutDataTypeStr=double
  rate_roll_pid_input1 : DataStoreMemory  DataStoreName=rate_roll_pid_input  ReadBeforeWriteMsg=warning  WriteAfterWriteMsg=warning  WriteAfterReadMsg=warning  InitialValue=rate_roll_pid_input  VectorParams1D=off  ShowAdditionalParam=off  OutDataTypeStr=double
  rate_roll_pid_integrator1 : DataStoreMemory  DataStoreName=rate_roll_pid_integrator  ReadBeforeWriteMsg=warning  WriteAfterWriteMsg=warning  WriteAfterReadMsg=warning  InitialValue=rate_roll_pid_integrator  VectorParams1D=off  ShowAdditionalParam=off  OutDataTypeStr=double
  rate_roll_pid_reset_filter1 : DataStoreMemory  DataStoreName=rate_roll_pid_reset_filter  ReadBeforeWriteMsg=warning  WriteAfterWriteMsg=warning  WriteAfterReadMsg=warning  InitialValue=rate_roll_pid_reset_filter  VectorParams1D=off  ShowAdditionalParam=off  OutDataTypeStr=double
  rate_target_ang_vel1 : DataStoreMemory  DataStoreName=rate_target_ang_vel  ReadBeforeWriteMsg=warning  WriteAfterWriteMsg=warning  WriteAfterReadMsg=warning  InitialValue=rate_target_ang_vel  VectorParams1D=off  ShowAdditionalParam=off  OutDataTypeStr=double
  rate_yaw_pid_derivative1 : DataStoreMemory  DataStoreName=rate_yaw_pid_derivative  ReadBeforeWriteMsg=warning  WriteAfterWriteMsg=warning  WriteAfterReadMsg=warning  InitialValue=rate_yaw_pid_derivative  VectorParams1D=off  ShowAdditionalParam=off  OutDataTypeStr=double
  rate_yaw_pid_input1 : DataStoreMemory  DataStoreName=rate_yaw_pid_input  ReadBeforeWriteMsg=warning  WriteAfterWriteMsg=warning  WriteAfterReadMsg=warning  InitialValue=rate_yaw_pid_input  VectorParams1D=off  ShowAdditionalParam=off  OutDataTypeStr=double
  rate_yaw_pid_integrator1 : DataStoreMemory  DataStoreName=rate_yaw_pid_integrator  ReadBeforeWriteMsg=warning  WriteAfterWriteMsg=warning  WriteAfterReadMsg=warning  InitialValue=rate_roll_pid_integrator  VectorParams1D=off  ShowAdditionalParam=off  OutDataTypeStr=double
  rate_yaw_pid_reset_filter1 : DataStoreMemory  DataStoreName=rate_yaw_pid_reset_filter  ReadBeforeWriteMsg=warning  WriteAfterWriteMsg=warning  WriteAfterReadMsg=warning  InitialValue=rate_yaw_pid_reset_filter  VectorParams1D=off  ShowAdditionalParam=off  OutDataTypeStr=double
  recalc_leash_xy1 : DataStoreMemory  DataStoreName=recalc_leash_xy  ReadBeforeWriteMsg=warning  WriteAfterWriteMsg=warning  WriteAfterReadMsg=warning  InitialValue=recalc_leash_xy  VectorParams1D=off  ShowAdditionalParam=off  OutDataTypeStr=double
  recalc_leash_z1 : DataStoreMemory  DataStoreName=recalc_leash_z  ReadBeforeWriteMsg=warning  WriteAfterWriteMsg=warning  WriteAfterReadMsg=warning  InitialValue=recalc_leash_z  ShowAdditionalParam=off  OutDataTypeStr=double
  reset_accel_to_lean_xy1 : DataStoreMemory  DataStoreName=reset_accel_to_lean_xy  ReadBeforeWriteMsg=warning  WriteAfterWriteMsg=warning  WriteAfterReadMsg=warning  InitialValue=reset_accel_to_lean_xy  VectorParams1D=off  ShowAdditionalParam=off  OutDataTypeStr=double
  reset_accel_to_throttle1 : DataStoreMemory  DataStoreName=reset_accel_to_throttle  ReadBeforeWriteMsg=warning  WriteAfterWriteMsg=warning  WriteAfterReadMsg=warning  InitialValue=reset_accel_to_throttle  VectorParams1D=off  ShowAdditionalParam=off  OutDataTypeStr=double
  reset_desired_vel_to_pos1 : DataStoreMemory  DataStoreName=reset_desired_vel_to_pos  ReadBeforeWriteMsg=warning  WriteAfterWriteMsg=warning  WriteAfterReadMsg=warning  InitialValue=reset_desired_vel_to_pos  VectorParams1D=off  ShowAdditionalParam=off  OutDataTypeStr=double
  reset_rate_to_accel_z1 : DataStoreMemory  DataStoreName=reset_rate_to_accel_z  ReadBeforeWriteMsg=warning  WriteAfterWriteMsg=warning  WriteAfterReadMsg=warning  InitialValue=reset_rate_to_accel_z  VectorParams1D=off  ShowAdditionalParam=off  OutDataTypeStr=double
  reverse1 : DataStoreMemory  DataStoreName=reverse  ReadBeforeWriteMsg=warning  WriteAfterWriteMsg=warning  WriteAfterReadMsg=warning  InitialValue=reverse  VectorParams1D=off  ShowAdditionalParam=off  OutDataTypeStr=double
  roll1 : DataStoreMemory  DataStoreName=roll  ReadBeforeWriteMsg=warning  WriteAfterWriteMsg=warning  WriteAfterReadMsg=warning  InitialValue=roll  ShowAdditionalParam=off  OutDataTypeStr=double
  rollComp1 : DataStoreMemory  DataStoreName=rollComp  ReadBeforeWriteMsg=warning  WriteAfterWriteMsg=warning  WriteAfterReadMsg=warning  InitialValue=rollComp  VectorParams1D=off  ShowAdditionalParam=off  OutDataTypeStr=double
  roll_factor1 : DataStoreMemory  DataStoreName=roll_factor  ReadBeforeWriteMsg=warning  WriteAfterWriteMsg=warning  WriteAfterReadMsg=warning  InitialValue=roll_factor  VectorParams1D=off  ShowAdditionalParam=off  OutDataTypeStr=double
  roll_ff_pitch1 : DataStoreMemory  DataStoreName=roll_ff_pitch  ReadBeforeWriteMsg=warning  WriteAfterWriteMsg=warning  WriteAfterReadMsg=warning  InitialValue=roll_ff_pitch  ShowAdditionalParam=off  OutDataTypeStr=double
  roll_ff_pitch_inint1 : DataStoreMemory  DataStoreName=roll_ff_pitch_inint  ReadBeforeWriteMsg=warning  WriteAfterWriteMsg=warning  WriteAfterReadMsg=warning  InitialValue=roll_ff_pitch_inint  VectorParams1D=off  ShowAdditionalParam=off  OutDataTypeStr=double
  roll_in1 : DataStoreMemory  DataStoreName=roll_in  ReadBeforeWriteMsg=warning  WriteAfterWriteMsg=warning  WriteAfterReadMsg=warning  InitialValue=roll_in  VectorParams1D=off  ShowAdditionalParam=off  OutDataTypeStr=double
  roll_limit_cd1 : DataStoreMemory  DataStoreName=roll_limit_cd  ReadBeforeWriteMsg=warning  WriteAfterWriteMsg=warning  WriteAfterReadMsg=warning  InitialValue=roll_limit_cd  ShowAdditionalParam=off  OutDataTypeStr=double
  roll_limit_cd_inint1 : DataStoreMemory  DataStoreName=roll_limit_cd_inint  ReadBeforeWriteMsg=warning  WriteAfterWriteMsg=warning  WriteAfterReadMsg=warning  InitialValue=roll_limit_cd_inint  ShowAdditionalParam=off  OutDataTypeStr=double
  roll_target1 : DataStoreMemory  DataStoreName=roll_target  ReadBeforeWriteMsg=warning  WriteAfterWriteMsg=warning  WriteAfterReadMsg=warning  InitialValue=roll_target  VectorParams1D=off  ShowAdditionalParam=off  OutDataTypeStr=double
  roll_target_pilot1 : DataStoreMemory  DataStoreName=roll_target_pilot  ReadBeforeWriteMsg=warning  WriteAfterWriteMsg=warning  WriteAfterReadMsg=warning  InitialValue=roll_target_pilot  VectorParams1D=off  ShowAdditionalParam=off  OutDataTypeStr=double
  rot_body_to_ned1 : DataStoreMemory  DataStoreName=rot_body_to_ned  ReadBeforeWriteMsg=warning  WriteAfterWriteMsg=warning  WriteAfterReadMsg=warning  InitialValue=rot_body_to_ned  VectorParams1D=off  ShowAdditionalParam=off  OutDataTypeStr=double
  scaling_speed1 : DataStoreMemory  DataStoreName=scaling_speed  ReadBeforeWriteMsg=warning  WriteAfterWriteMsg=warning  WriteAfterReadMsg=warning  InitialValue=scaling_speed  ShowAdditionalParam=off  OutDataTypeStr=double
  slew_yaw1 : DataStoreMemory  DataStoreName=slew_yaw  ReadBeforeWriteMsg=warning  WriteAfterWriteMsg=warning  WriteAfterReadMsg=warning  InitialValue=slew_yaw  VectorParams1D=off  ShowAdditionalParam=off  OutDataTypeStr=double
  smoothed_airspeed1 : DataStoreMemory  DataStoreName=smoothed_airspeed  ReadBeforeWriteMsg=warning  WriteAfterWriteMsg=warning  WriteAfterReadMsg=warning  InitialValue=smoothed_airspeed  ShowAdditionalParam=off  OutDataTypeStr=double
  spdCompFiltOmega1 : DataStoreMemory  DataStoreName=spdCompFiltOmega  ReadBeforeWriteMsg=warning  WriteAfterWriteMsg=warning  WriteAfterReadMsg=warning  InitialValue=spdCompFiltOmega  VectorParams1D=off  ShowAdditionalParam=off  OutDataTypeStr=double
  spdWeight1 : DataStoreMemory  DataStoreName=spdWeight  ReadBeforeWriteMsg=warning  WriteAfterWriteMsg=warning  WriteAfterReadMsg=warning  InitialValue=spdWeight  VectorParams1D=off  ShowAdditionalParam=off  OutDataTypeStr=double
  spdWeight_inint : DataStoreMemory  DataStoreName=spdWeight_inint  ReadBeforeWriteMsg=warning  WriteAfterWriteMsg=warning  WriteAfterReadMsg=warning  InitialValue=spdWeight_inint  VectorParams1D=off  ShowAdditionalParam=off  OutDataTypeStr=double
  tail_tilt1 : DataStoreMemory  DataStoreName=tail_tilt  ReadBeforeWriteMsg=warning  WriteAfterWriteMsg=warning  WriteAfterReadMsg=warning  InitialValue=tail_tilt  VectorParams1D=off  ShowAdditionalParam=off  OutDataTypeStr=double
  tail_tilt_c2p1 : DataStoreMemory  DataStoreName=tail_tilt_c2p  ReadBeforeWriteMsg=warning  WriteAfterWriteMsg=warning  WriteAfterReadMsg=warning  InitialValue=tail_tilt_c2p  VectorParams1D=off  ShowAdditionalParam=off  OutDataTypeStr=double
  tail_tilt_p2c1 : DataStoreMemory  DataStoreName=tail_tilt_p2c  ReadBeforeWriteMsg=warning  WriteAfterWriteMsg=warning  WriteAfterReadMsg=warning  InitialValue=tail_tilt_p2c  VectorParams1D=off  ShowAdditionalParam=off  OutDataTypeStr=double
  tail_tilt_rate1 : DataStoreMemory  DataStoreName=tail_tilt_rate  ReadBeforeWriteMsg=warning  WriteAfterWriteMsg=warning  WriteAfterReadMsg=warning  InitialValue=tail_tilt_rate  VectorParams1D=off  ShowAdditionalParam=off  OutDataTypeStr=double
  take_off_land : DataStoreMemory  DataStoreName=take_off_land  ReadBeforeWriteMsg=warning  WriteAfterWriteMsg=warning  WriteAfterReadMsg=warning  InitialValue=take_off_land  VectorParams1D=off  ShowAdditionalParam=off  OutDataTypeStr=double
  target_bearing_cd1 : DataStoreMemory  DataStoreName=target_bearing_cd  ReadBeforeWriteMsg=warning  WriteAfterWriteMsg=warning  WriteAfterReadMsg=warning  InitialValue=target_bearing_cd  VectorParams1D=off  ShowAdditionalParam=off  OutDataTypeStr=double
  target_yaw_rate1 : DataStoreMemory  DataStoreName=target_yaw_rate  ReadBeforeWriteMsg=warning  WriteAfterWriteMsg=warning  WriteAfterReadMsg=warning  InitialValue=target_yaw_rate  VectorParams1D=off  ShowAdditionalParam=off  OutDataTypeStr=double
  thrDamp1 : DataStoreMemory  DataStoreName=thrDamp  ReadBeforeWriteMsg=warning  WriteAfterWriteMsg=warning  WriteAfterReadMsg=warning  InitialValue=thrDamp  VectorParams1D=off  ShowAdditionalParam=off  OutDataTypeStr=double
  thr_out_min : DataStoreMemory  DataStoreName=thr_out_min  ReadBeforeWriteMsg=warning  WriteAfterWriteMsg=warning  WriteAfterReadMsg=warning  InitialValue=thr_out_min  VectorParams1D=off  ShowAdditionalParam=off  OutDataTypeStr=double
  thr_out_min_c2p : DataStoreMemory  DataStoreName=thr_out_min_c2p  ReadBeforeWriteMsg=warning  WriteAfterWriteMsg=warning  WriteAfterReadMsg=warning  InitialValue=thr_out_min_c2p  VectorParams1D=off  ShowAdditionalParam=off  OutDataTypeStr=double
  thr_out_min_inint : DataStoreMemory  DataStoreName=thr_out_min_inint  ReadBeforeWriteMsg=warning  WriteAfterWriteMsg=warning  WriteAfterReadMsg=warning  InitialValue=thr_out_min_inint  VectorParams1D=off  ShowAdditionalParam=off  OutDataTypeStr=double
  throttle_avg_max1 : DataStoreMemory  DataStoreName=throttle_avg_max  ReadBeforeWriteMsg=warning  WriteAfterWriteMsg=warning  WriteAfterReadMsg=warning  InitialValue=throttle_avg_max  VectorParams1D=off  ShowAdditionalParam=off  OutDataTypeStr=double
  throttle_cruise1 : DataStoreMemory  DataStoreName=throttle_cruise  ReadBeforeWriteMsg=warning  WriteAfterWriteMsg=warning  WriteAfterReadMsg=warning  InitialValue=throttle_cruise  VectorParams1D=off  ShowAdditionalParam=off  OutDataTypeStr=double
  throttle_cutoff_frequency1 : DataStoreMemory  DataStoreName=throttle_cutoff_frequency  ReadBeforeWriteMsg=warning  WriteAfterWriteMsg=warning  WriteAfterReadMsg=warning  InitialValue=throttle_cutoff_frequency  VectorParams1D=off  ShowAdditionalParam=off  OutDataTypeStr=double
  throttle_dem1 : DataStoreMemory  DataStoreName=throttle_dem  ReadBeforeWriteMsg=warning  WriteAfterWriteMsg=warning  WriteAfterReadMsg=warning  InitialValue=throttle_dem  VectorParams1D=off  ShowAdditionalParam=off  OutDataTypeStr=double
  throttle_filter1 : DataStoreMemory  DataStoreName=throttle_filter  ReadBeforeWriteMsg=warning  WriteAfterWriteMsg=warning  WriteAfterReadMsg=warning  InitialValue=throttle_filter  VectorParams1D=off  ShowAdditionalParam=off  OutDataTypeStr=double
  throttle_ground : DataStoreMemory  DataStoreName=throttle_ground  ReadBeforeWriteMsg=warning  WriteAfterWriteMsg=warning  WriteAfterReadMsg=warning  InitialValue=throttle_ground  VectorParams1D=off  ShowAdditionalParam=off  OutDataTypeStr=double
  throttle_hover1 : DataStoreMemory  DataStoreName=throttle_hover  ReadBeforeWriteMsg=warning  WriteAfterWriteMsg=warning  WriteAfterReadMsg=warning  InitialValue=throttle_hover  VectorParams1D=off  ShowAdditionalParam=off  OutDataTypeStr=double
  throttle_in1 : DataStoreMemory  DataStoreName=throttle_in  ReadBeforeWriteMsg=warning  WriteAfterWriteMsg=warning  WriteAfterReadMsg=warning  InitialValue=throttle_in  VectorParams1D=off  ShowAdditionalParam=off  OutDataTypeStr=double
  throttle_lower1 : DataStoreMemory  DataStoreName=throttle_lower  ReadBeforeWriteMsg=warning  WriteAfterWriteMsg=warning  WriteAfterReadMsg=warning  InitialValue=throttle_lower  VectorParams1D=off  ShowAdditionalParam=off  OutDataTypeStr=double
  throttle_max1 : DataStoreMemory  DataStoreName=throttle_max  ReadBeforeWriteMsg=warning  WriteAfterWriteMsg=warning  WriteAfterReadMsg=warning  InitialValue=throttle_max  VectorParams1D=off  ShowAdditionalParam=off  OutDataTypeStr=double
  throttle_min1 : DataStoreMemory  DataStoreName=throttle_min  ReadBeforeWriteMsg=warning  WriteAfterWriteMsg=warning  WriteAfterReadMsg=warning  InitialValue=throttle_min  VectorParams1D=off  ShowAdditionalParam=off  OutDataTypeStr=double
  throttle_off_rate : DataStoreMemory  DataStoreName=throttle_off_rate  ReadBeforeWriteMsg=warning  WriteAfterWriteMsg=warning  WriteAfterReadMsg=warning  InitialValue=throttle_off_rate  VectorParams1D=off  ShowAdditionalParam=off  OutDataTypeStr=double
  throttle_rpy_mix1 : DataStoreMemory  DataStoreName=throttle_rpy_mix  ReadBeforeWriteMsg=warning  WriteAfterWriteMsg=warning  WriteAfterReadMsg=warning  InitialValue=throttle_rpy_mix  VectorParams1D=off  ShowAdditionalParam=off  OutDataTypeStr=double
  throttle_rpy_mix_desired1 : DataStoreMemory  DataStoreName=throttle_rpy_mix_desired  ReadBeforeWriteMsg=warning  WriteAfterWriteMsg=warning  WriteAfterReadMsg=warning  InitialValue=throttle_rpy_mix_desired  VectorParams1D=off  ShowAdditionalParam=off  OutDataTypeStr=double
  throttle_slewrate1 : DataStoreMemory  DataStoreName=throttle_slewrate  ReadBeforeWriteMsg=warning  WriteAfterWriteMsg=warning  WriteAfterReadMsg=warning  InitialValue=throttle_slewrate  VectorParams1D=off  ShowAdditionalParam=off  OutDataTypeStr=double
  throttle_thrust_max1 : DataStoreMemory  DataStoreName=throttle_thrust_max  ReadBeforeWriteMsg=warning  WriteAfterWriteMsg=warning  WriteAfterReadMsg=warning  InitialValue=throttle_thrust_max  VectorParams1D=off  ShowAdditionalParam=off  OutDataTypeStr=double
  throttle_upper1 : DataStoreMemory  DataStoreName=throttle_upper  ReadBeforeWriteMsg=warning  WriteAfterWriteMsg=warning  WriteAfterReadMsg=warning  InitialValue=throttle_upper  VectorParams1D=off  ShowAdditionalParam=off  OutDataTypeStr=double
  thrust_boost1 : DataStoreMemory  DataStoreName=thrust_boost  ReadBeforeWriteMsg=warning  WriteAfterWriteMsg=warning  WriteAfterReadMsg=warning  InitialValue=thrust_boost  VectorParams1D=off  ShowAdditionalParam=off  OutDataTypeStr=double
  thrust_boost_ratio1 : DataStoreMemory  DataStoreName=thrust_boost_ratio  ReadBeforeWriteMsg=warning  WriteAfterWriteMsg=warning  WriteAfterReadMsg=warning  InitialValue=thrust_boost_ratio  VectorParams1D=off  ShowAdditionalParam=off  OutDataTypeStr=double
  thrust_error_angle1 : DataStoreMemory  DataStoreName=thrust_error_angle  ReadBeforeWriteMsg=warning  WriteAfterWriteMsg=warning  WriteAfterReadMsg=warning  InitialValue=thrust_error_angle  VectorParams1D=off  ShowAdditionalParam=off  OutDataTypeStr=double
  thrust_rpyt_out1 : DataStoreMemory  DataStoreName=thrust_rpyt_out  ReadBeforeWriteMsg=warning  WriteAfterWriteMsg=warning  WriteAfterReadMsg=warning  InitialValue=thrust_rpyt_out  VectorParams1D=off  ShowAdditionalParam=off  OutDataTypeStr=double
  thrust_slew_time1 : DataStoreMemory  DataStoreName=thrust_slew_time  ReadBeforeWriteMsg=warning  WriteAfterWriteMsg=warning  WriteAfterReadMsg=warning  InitialValue=thrust_slew_time  VectorParams1D=off  ShowAdditionalParam=off  OutDataTypeStr=double
  timeConstant1 : DataStoreMemory  DataStoreName=timeConstant  ReadBeforeWriteMsg=warning  WriteAfterWriteMsg=warning  WriteAfterReadMsg=warning  InitialValue=timeConstant  VectorParams1D=off  ShowAdditionalParam=off  OutDataTypeStr=double
  use_desvel_ff_z1 : DataStoreMemory  DataStoreName=use_desvel_ff_z  ReadBeforeWriteMsg=warning  WriteAfterWriteMsg=warning  WriteAfterReadMsg=warning  InitialValue=use_desvel_ff_z  VectorParams1D=off  ShowAdditionalParam=off  OutDataTypeStr=double
  use_sqrt_controller1 : DataStoreMemory  DataStoreName=use_sqrt_controller  ReadBeforeWriteMsg=warning  WriteAfterWriteMsg=warning  WriteAfterReadMsg=warning  InitialValue=use_sqrt_controller  ShowAdditionalParam=off  OutDataTypeStr=double
  vdot_filter1 : DataStoreMemory  DataStoreName=vdot_filter  ReadBeforeWriteMsg=warning  WriteAfterWriteMsg=warning  WriteAfterReadMsg=warning  InitialValue=vdot_filter  ShowAdditionalParam=off  OutDataTypeStr=double
  vel_desired1 : DataStoreMemory  DataStoreName=vel_desired  ReadBeforeWriteMsg=warning  WriteAfterWriteMsg=warning  WriteAfterReadMsg=warning  InitialValue=vel_desired  VectorParams1D=off  ShowAdditionalParam=off  OutDataTypeStr=double
  vel_dot1 : DataStoreMemory  DataStoreName=vel_dot  ReadBeforeWriteMsg=warning  WriteAfterWriteMsg=warning  WriteAfterReadMsg=warning  InitialValue=vel_dot  VectorParams1D=off  ShowAdditionalParam=off  OutDataTypeStr=double
  vel_error1 : DataStoreMemory  DataStoreName=vel_error  ReadBeforeWriteMsg=warning  WriteAfterWriteMsg=warning  WriteAfterReadMsg=warning  InitialValue=vel_error  VectorParams1D=off  ShowAdditionalParam=off  OutDataTypeStr=double
  vel_error_input1 : DataStoreMemory  DataStoreName=vel_error_input  ReadBeforeWriteMsg=warning  WriteAfterWriteMsg=warning  WriteAfterReadMsg=warning  InitialValue=vel_error_input  VectorParams1D=off  ShowAdditionalParam=off  OutDataTypeStr=double
  vel_forward_gain1 : DataStoreMemory  DataStoreName=vel_forward_gain  ReadBeforeWriteMsg=warning  WriteAfterWriteMsg=warning  WriteAfterReadMsg=warning  InitialValue=vel_forward_gain  VectorParams1D=off  ShowAdditionalParam=off  OutDataTypeStr=double
  vel_forward_integrator : DataStoreMemory  DataStoreName=vel_forward_integrator  ReadBeforeWriteMsg=warning  WriteAfterWriteMsg=warning  WriteAfterReadMsg=warning  InitialValue=vel_forward_integrator  VectorParams1D=off  ShowAdditionalParam=off  OutDataTypeStr=double
  vel_forward_last_pct1 : DataStoreMemory  DataStoreName=vel_forward_last_pct  ReadBeforeWriteMsg=warning  WriteAfterWriteMsg=warning  WriteAfterReadMsg=warning  InitialValue=vel_forward_last_pct  VectorParams1D=off  ShowAdditionalParam=off  OutDataTypeStr=double
  vel_forward_min_pitch1 : DataStoreMemory  DataStoreName=vel_forward_min_pitch  ReadBeforeWriteMsg=warning  WriteAfterWriteMsg=warning  WriteAfterReadMsg=warning  InitialValue=vel_forward_min_pitch  VectorParams1D=off  ShowAdditionalParam=off  OutDataTypeStr=double
  vel_forward_tail_tilt_max1 : DataStoreMemory  DataStoreName=vel_forward_tail_tilt_max  ReadBeforeWriteMsg=warning  WriteAfterWriteMsg=warning  WriteAfterReadMsg=warning  InitialValue=vel_forward_tail_tilt_max  VectorParams1D=off  ShowAdditionalParam=off  OutDataTypeStr=double
  vel_last1 : DataStoreMemory  DataStoreName=vel_last  ReadBeforeWriteMsg=warning  WriteAfterWriteMsg=warning  WriteAfterReadMsg=warning  InitialValue=vel_last  VectorParams1D=off  ShowAdditionalParam=off  OutDataTypeStr=double
  vel_target1 : DataStoreMemory  DataStoreName=vel_target  ReadBeforeWriteMsg=warning  WriteAfterWriteMsg=warning  WriteAfterReadMsg=warning  InitialValue=vel_target  VectorParams1D=off  ShowAdditionalParam=off  OutDataTypeStr=double
  vertAccLim1 : DataStoreMemory  DataStoreName=vertAccLim  ReadBeforeWriteMsg=warning  WriteAfterWriteMsg=warning  WriteAfterReadMsg=warning  InitialValue=vertAccLim  VectorParams1D=off  ShowAdditionalParam=off  OutDataTypeStr=double
  weathervane_gain1 : DataStoreMemory  DataStoreName=weathervane_gain  ReadBeforeWriteMsg=warning  WriteAfterWriteMsg=warning  WriteAfterReadMsg=warning  InitialValue=weathervane_gain  VectorParams1D=off  ShowAdditionalParam=off  OutDataTypeStr=double
  weathervane_last_output1 : DataStoreMemory  DataStoreName=weathervane_last_output  ReadBeforeWriteMsg=warning  WriteAfterWriteMsg=warning  WriteAfterReadMsg=warning  InitialValue=weathervane_last_output  VectorParams1D=off  ShowAdditionalParam=off  OutDataTypeStr=double
  weathervane_min_roll1 : DataStoreMemory  DataStoreName=weathervane_min_roll  ReadBeforeWriteMsg=warning  WriteAfterWriteMsg=warning  WriteAfterReadMsg=warning  InitialValue=weathervane_min_roll  VectorParams1D=off  ShowAdditionalParam=off  OutDataTypeStr=double
  yaw1 : DataStoreMemory  DataStoreName=yaw  ReadBeforeWriteMsg=warning  WriteAfterWriteMsg=warning  WriteAfterReadMsg=warning  InitialValue=yaw  VectorParams1D=off  ShowAdditionalParam=off  OutDataTypeStr=double
  yaw_factor1 : DataStoreMemory  DataStoreName=yaw_factor  ReadBeforeWriteMsg=warning  WriteAfterWriteMsg=warning  WriteAfterReadMsg=warning  InitialValue=yaw_factor  VectorParams1D=off  ShowAdditionalParam=off  OutDataTypeStr=double
  yaw_headroom1 : DataStoreMemory  DataStoreName=yaw_headroom  ReadBeforeWriteMsg=warning  WriteAfterWriteMsg=warning  WriteAfterReadMsg=warning  InitialValue=yaw_headroom  VectorParams1D=off  ShowAdditionalParam=off  OutDataTypeStr=double
  yaw_in1 : DataStoreMemory  DataStoreName=yaw_in  ReadBeforeWriteMsg=warning  WriteAfterWriteMsg=warning  WriteAfterReadMsg=warning  InitialValue=yaw_in  VectorParams1D=off  ShowAdditionalParam=off  OutDataTypeStr=double
  yaw_in_max : DataStoreMemory  DataStoreName=yaw_in_max  ReadBeforeWriteMsg=warning  WriteAfterWriteMsg=warning  WriteAfterReadMsg=warning  InitialValue=yaw_in_max  VectorParams1D=off  ShowAdditionalParam=off  OutDataTypeStr=double
  yaw_max_c2p1 : DataStoreMemory  DataStoreName=yaw_max_c2p  ReadBeforeWriteMsg=warning  WriteAfterWriteMsg=warning  WriteAfterReadMsg=warning  InitialValue=yaw_max_c2p  VectorParams1D=off  ShowAdditionalParam=off  OutDataTypeStr=double
  yaw_rate_max1 : DataStoreMemory  DataStoreName=yaw_rate_max  ReadBeforeWriteMsg=warning  WriteAfterWriteMsg=warning  WriteAfterReadMsg=warning  InitialValue=yaw_rate_max  VectorParams1D=off  ShowAdditionalParam=off  OutDataTypeStr=double
  z_accel_meas1 : DataStoreMemory  DataStoreName=z_accel_meas  ReadBeforeWriteMsg=warning  WriteAfterWriteMsg=warning  WriteAfterReadMsg=warning  InitialValue=z_accel_meas  VectorParams1D=off  ShowAdditionalParam=off  OutDataTypeStr=double
  Out1 : Outport  OutDataTypeStr=Bus: BUS_CTRL_Sevro_pwm
  wires:
  Data Store Read140/1 -> Scope168/1
  Data Store Read142/1 -> Scope174/1
  Constant30/1 -> Mux4/3
  Data Store Read46/1 -> Gain26/1
  6DOF (Euler Angles)2/6(p,q,r) -> [wb]
  Demux45/1 -> Hypot3/1
  [Xe] -> Scope136/1, To Workspace3/1
  Demux45/2 -> Hypot3/2
  Inertial to Body5/1 -> [Vwb]
  Demux44/1 -> Hypot2/1
  [Ve] -> Sum1/1
  Data Store Read71/1 -> Scope153/1
  Location_offset1/1(current_loc) -> get_vector_xy_from_origin_NE1/1(loc), Demux42/1, To Workspace2/1, Data Store Write41/1
  Constant37/1 -> Data Store Write33/1
  6DOF (Euler Angles)2/2(Xe) -> [Xe]
  Data Store Read125/1 -> Scope132/1
  Demux42/2 -> Scope85/1
  Constant38/1 -> Location_offset1/1(center_WP)
  Sine Wave1/1 -> Scope146/1
  Demux46/3 -> Terminator10/1
  Demux38/2 -> Scope154/2
  gn3/1 -> Gravity in Earth Axes2/1
  Demux15/3 -> Scope155/3
  Demux37/3 -> Data Store Write52/1
  Demux36/2 -> Scope100/1
  Data Store Read67/1 -> Scope148/2, Scope147/1
  Atan3/1 -> [yaw_gps]
  "Incidence, Sideslip & Airspeed3"/2 -> Gain37/1  "Beta"
  Data Store Read41/1 -> Scope88/1
  Add7/1 -> Demux/1, Scope15/1, Delay7/1
  Gain28/1 -> Data Store Write50/1
  Data Store Read62/1 -> Scope130/1
  Data Store Read117/1 -> Gain31/1
  Demux37/1 -> Data Store Write51/1
  Hypot2/1 -> Data Store Write32/1
  Demux40/1 -> Scope158/1
  Constant28/1 -> Data Store Write54/1
  Add2/1 -> Demux22/1
  6DOF (Euler Angles)2/1(Ve) -> [Ve]
  Gain14/1 -> Scope140/1
  Demux15/4 -> Scope155/4
  Data Store Read126/1 -> Scope145/1, Demux14/1
  Constant35/1 -> Data Store Write31/1
  Data Store Read121/1 -> Scope121/2, Scope142/1
  Data Store Read60/1 -> Display1/1
  Add5/1 -> Scope119/1, Delay6/1
  Data Store Read109/1 -> Scope18/1, Scope141/1
  Demux22/3 -> Data Store Write44/1
  Demux41/3 -> Terminator2/1
  Gain27/1 -> MATLAB Function1/11(alt)
  Demux21/1 -> Terminator/1
  Data Store Read137/1 -> Scope169/1
  Gain36/1 -> Scope86/1
  Demux36/1 -> Scope99/1
  Gain45/1 -> Data Store Write61/1
  Gain35/1 -> Scope167/2, Scope166/1
  Data Store Read113/1 -> Scope122/1, Scope102/1
  Constant25/1 -> Data Store Write43/1
  Demux43/1 -> Scope110/1
  Data Store Read136/1 -> Scope160/1
  Data Store Read69/1 -> Scope148/1
  Data Store Read63/1 -> Scope129/1
  Data Store Read37/1 -> Scope80/1
  Demux22/1 -> Data Store Write40/1
  Demux12/1 -> Terminator6/1
  Constant12/1 -> Mux4/1
  Data Store Read135/1 -> Scope18/2, Scope161/1
  Demux10/1 -> Data Store Write56/1
  Demux14/4 -> Scope143/4
  Data Store Read7/1 -> Gain1/1
  Demux15/1 -> Scope155/1
  Constant34/1 -> Data Store Write37/1
  Demux16/2 -> Scope150/2
  Hypot3/1 -> Derivative1/1, Scope138/1, Scope135/1
  Demux13/2 -> Scope95/2
  Data Store Read40/1 -> Gain41/1
  Constant31/1 -> Data Store Write36/1
  Data Store Read123/1 -> Scope115/1
  Constant41/1 -> Data Store Write53/1
  Delay7/1 -> 6DOF (Euler Angles)2/2(Moments)
  Data Store Read59/1 -> Scope128/1
  Demux12/3 -> Gain44/1, Gain28/1
  Demux39/3 -> Data Store Write49/1
  Demux39/1 -> Mux3/1
  Data Store Read108/1 -> Demux9/1
  6DOF (Euler Angles)2/8(Ab) -> [Abb]
  "Incidence, Sideslip & Airspeed2"/2(Beta) -> MATLAB Function1/9(beta), Gain35/1  "Beta"
  Data Store Read53/1 -> Gain46/1
  Demux13/3 -> Scope124/2, Scope95/3
  gn4/1 -> Inertial to Body6/2
  Gravity in Earth Axes2/1 -> Inertial to Body4/2
  Data Store Read134/1 -> Gain2/1
  Gain29/1 -> Add2/2
  "Incidence, Sideslip & Airspeed2"/3(V) -> [V]
  Data Store Read118/1 -> Gain32/1
  Data Store Read143/1 -> Gain38/1
  Data Store Read122/1 -> Scope127/1
  Gain47/1 -> Scope117/2
  Demux19/1 -> Scope151/1
  [euler] -> Demux37/1
  Demux14/1 -> Scope143/1
  Mux5/1 -> Gain14/1
  Demux37/2 -> Data Store Write38/1
  Demux40/2 -> Scope158/2
  Demux16/1 -> Scope150/1
  Add1/1 -> 6DOF (Euler Angles)2/1(Forces), Scope144/1
  Data Store Read110/1 -> Scope122/2, Scope60/1
  Gain31/1 -> Scope175/1
  Gain1/1 -> Scope163/1
  Constant27/1 -> Data Store Write35/1
  Data Store Read65/1 -> Demux45/1, Scope134/1
  Data Store Read138/1 -> Scope165/1
  Demux40/3 -> Scope158/3
  Delay6/1 -> Add1/1
  Demux23/2 -> Scope157/2
  Demux47/3 -> Terminator11/1
  Constant13/1 -> Mux4/2
  "Incidence, Sideslip & Airspeed2"/1(Alpha) -> MATLAB Function1/8(alpha), Gain34/1  "alpha"
  Demux44/2 -> Hypot2/2
  Demux23/1 -> Scope157/1
  [Vb] -> "Incidence, Sideslip & Airspeed3"/1
  [Xe] -> Demux41/1, Scope125/1, Demux12/1
  "Incidence, Sideslip & Airspeed3"/3 -> Scope71/1
  Gain2/1 -> Scope163/2
  Data Store Read111/1 -> MATLAB Function1/1(k_rudder), Gain30/1
  Gain41/1 -> Scope114/1, Scope87/2
  Constant40/1 -> Data Store Write47/1
  Demux9/1 -> Scope116/1
  Demux46/1 -> Atan4/2
  6DOF (Euler Angles)2/4(DCM) -> [DCM_be]
  Data Store Read131/1 -> Demux40/1
  Demux19/2 -> Scope151/2
  [yaw_w] -> Mux5/2
  Demux46/2 -> Atan4/1
  Data Store Read55/1 -> Scope118/1
  Data Store Read36/1 -> Gain39/1
  Demux22/2 -> Data Store Write39/1
  Data Store Read68/1 -> Gain36/1
  Constant36/1 -> Demux43/1, get_vector_xy_from_origin_NE1/2(loc_origin)
  Demux9/2 -> Scope116/2
  Gain38/1 -> Scope117/1, Scope73/2
  [yaw_gps] -> Mux5/3
  Data Store Read130/1 -> Demux23/1
  Data Store Read120/1 -> Demux13/1
  [Xe] -> Demux21/1
  Demux20/1 -> MATLAB Function1/5(wx)
  Gain43/1 -> Scope92/1
  Data Store Read56/1 -> Scope65/1
  Inertial to Body6/1 -> Gain29/1
  Data Store Read141/1 -> Scope172/1
  Gain44/1 -> Data Store Write59/1
  Gain30/1 -> Scope167/1
  Data Store Read6/1 -> Scope1/1
  Demux13/1 -> Scope95/1
  Derivative1/1 -> Scope138/2, Scope137/1
  Demux38/3 -> Scope154/3
  Demux21/3 -> Gain27/1
  Constant1/1 -> Data Store Write4/1
  "Incidence, Sideslip & Airspeed3"/1 -> Gain49/1  "alpha"
  Gain32/1 -> Scope177/1
  get_vector_xy_from_origin_NE1/1(vec_ne) -> Demux36/1
  Data Store Read38/1 -> Gain40/1
  Data Store Read70/1 -> Scope149/1
  Data Store Read133/1 -> Scope96/1
  Data Store Read128/1 -> Demux19/1
  Data Store Read57/1 -> Scope133/1
  Demux14/2 -> Scope143/2
  [DCM_be] -> Inertial to Body5/1
  Data Store Read112/1 -> MATLAB Function1/2(k_aileron), Scope173/1
  Demux20/2 -> MATLAB Function1/6(wy)
  Data Store Read64/1 -> Scope131/1
  Data Store Read129/1 -> Demux38/1
  [wb] -> Demux10/1
  Constant29/1 -> Data Store Write60/1
  Gain48/1 -> Scope93/1
  Demux16/3 -> Scope150/3
  6DOF (Euler Angles)2/7(pdot,qdot,rdot) -> Terminator8/1
  Sum1/1 -> Demux46/1, Demux44/1, Scope139/1, Inertial to Body5/2  "Vwe"
  Data Store Read43/1 -> Scope162/1
  Data Store Read139/1 -> Scope171/1
  [wb] -> Demux20/1
  [DCM_be] -> Inertial to Body6/1
  [Ve] -> Scope152/1, Demux47/1, Demux39/1, Gain45/1
  Data Store Read39/1 -> Gain42/1
  Data Store Read124/1 -> Scope123/1
  Demux23/3 -> Scope121/1, Scope157/3
  Data Store Read127/1 -> Demux16/1
  Data Store Read119/1 -> Gain33/1
  Demux14/3 -> Scope143/3
  Demux39/2 -> Mux3/2
  Data Store Read132/1 -> Scope159/1
  Constant39/1 -> Data Store Write46/1
  Demux19/3 -> Scope124/1, Scope151/3
  Demux43/2 -> Scope113/1
  Data Store Read50/1 -> Scope98/1
  Mux3/1 -> Data Store Write42/1
  Constant32/1 -> Data Store Write45/1
  Demux38/1 -> Scope154/1
  6DOF (Euler Angles)2/5(Vb) -> [Vb]
  Demux12/2 -> Terminator7/1
  Data Store Read66/1 -> Mux5/1
  Data Store Read42/1 -> Scope88/2
  Demux41/1 -> Delay4/1
  Data Store Read114/1 -> MATLAB Function1/3(k_throttle), Scope179/1
  [Abb] -> Add2/1
  [Vwb] -> "Incidence, Sideslip & Airspeed2"/1(Vb)
  Data Store Read74/1 -> Gain48/1
  Gain39/1 -> Scope73/1
  Data Store Read48/1 -> Scope97/1, Demux15/1
  Data Store Read107/1 -> Gain43/1
  Gain34/1 -> Scope164/1
  Demux44/3 -> Terminator9/1
  Inertial to Body4/1 -> Scope120/1, Add1/2
  Delay5/1 -> Scope100/2, Location_offset1/3(ofs_east)
  Gain26/1 -> Scope170/2
  Data Store Read116/1 -> MATLAB Function1/4(k_elevator), Scope66/1
  [DCM_be] -> Inertial to Body4/1
  Gain49/1 -> Scope67/1
  Demux20/3 -> MATLAB Function1/7(wz)
  Constant33/1 -> Data Store Write48/1
  Data Store Read45/1 -> Scope176/2
  Demux47/1 -> Atan3/2
  Data Store Read54/1 -> Gain47/1
  Gain40/1 -> Scope72/1
  Demux10/2 -> Data Store Write57/1
  Gain37/1 -> Scope68/1
  Demux15/2 -> Scope155/2
  Data Store Read/1 -> Scope2/1
  Gain33/1 -> Scope178/1
  Data Store Read34/1 -> Scope170/1
  Demux47/2 -> Atan3/1
  Gain42/1 -> Scope87/1
  Demux41/2 -> Delay5/1
  Atan4/1 -> [yaw_w]
  Demux42/1 -> Scope58/1
  Gain46/1 -> Scope114/2
  Constant14/1 -> Data Store Write55/1
  Demux10/3 -> Data Store Write58/1
  Demux21/2 -> Terminator1/1
  Data Store Read44/1 -> Scope176/1
  Delay4/1 -> Location_offset1/2(ofs_north), Scope99/2
  6DOF (Euler Angles)2/3(Euler) -> [euler]
  Mux4/1 -> Sum1/2
  Constant26/1 -> Data Store Write34/1
  Data Store Read58/1 -> Scope126/1
  Data Store Read150/1 -> Scope83/3  "I"
  Data Store Read79/1 -> Scope83/2, Scope3/1  "D"
  Data Store Read1/1 -> Scope83/1, Scope54/1  "P"
  Data Store Read151/1 -> Scope83/4
  Gain3/1 -> Scope81/1
  Data Store Read83/1 -> Gain3/1
  Add4/1 -> Gain85/1
  Data Store Read149/1 -> Gain79/1
  Gain84/1 -> Add3/1
  Data Store Read5/1 -> Scope6/1
  Data Store Read8/1 -> Scope7/1
  Gain76/1 -> Scope9/1
  Data Store Read144/1 -> Gain76/1
  Data Store Read11/1 -> Gain83/1
  Data Store Read147/1 -> Gain78/1
  Gain77/1 -> Scope9/3
  Add/1 -> Gain84/1
  Gain83/1 -> Scope8/1, Add/1  "P"
  Gain79/1 -> Scope10/3
  Data Store Read166/1 -> Add4/1, Add3/2
  Gain85/1 -> Scope8/4
  Data Store Read148/1 -> Scope10/2
  Gain72/1 -> Scope8/2, Add/2  "D"
  Data Store Read10/1 -> Scope8/3, Add/3  "I"
  Data Store Read145/1 -> Scope9/2
  Data Store Read146/1 -> Gain77/1
  Data Store Read167/1 -> Add4/2, Scope78/2
  Gain78/1 -> Scope10/1
  Data Store Read9/1 -> Gain72/1
  Data Store Read4/1 -> Scope5/1
  Add3/1 -> Scope78/1
  Demux2/2 -> Scope12/2
  Data Store Read13/1 -> Demux2/1
  Demux1/3 -> Scope13/1
  Demux1/2 -> Scope12/1
  Demux1/1 -> Scope11/1
  Demux2/1 -> Scope11/2
  Demux1/4 -> Scope14/1
  Demux2/4 -> Scope14/2
  Demux2/3 -> Scope13/2
  MATLAB Function/1(PWM_n) -> Demux1/1
  Data Store Read12/1 -> MATLAB Function/1(PWM)
  Data Store Read14/1 -> Scope16/2
  Demux/2 -> Scope16/1
  Data Type Conversion7/1 -> ?  "gyro_z"
  Data Type Conversion5/1 -> ?  "gyro_x"
  Data Type Conversion10/1 -> ?  "accel_z"
  Data Type Conversion9/1 -> ?  "accel_y"
  Bus Selector1/4 -> Data Type Conversion11/1  "<alt>"
  Data Type Conversion1/1 -> Data Store Write2/6  "rolld"
  Data Type Conversion11/1 -> Data Store Write2/8  "NAV_alt"
  input_euler_angle_roll_pitch_euler_rate_yaw4/3(k_rudder_o) -> Bus Assignment/4  "k_rudder"
  Bus Selector1/1 -> Data Type Conversion/1  "<pitchd>"
  input_euler_angle_roll_pitch_euler_rate_yaw4/5(k_aileronR_o) -> Bus Assignment/6  "k_rudderR"
  input_euler_angle_roll_pitch_euler_rate_yaw4/9(k_flap_o) -> Bus Assignment/10  "k_flap"
  input_euler_angle_roll_pitch_euler_rate_yaw4/4(k_aileronL_o) -> Bus Assignment/5  "k_rudderL"
  input_euler_angle_roll_pitch_euler_rate_yaw4/2(k_elevator_o) -> Bus Assignment/3  "k_elevator"
  Data Type Conversion2/1 -> Data Store Write2/7  "yawd"
  Bus Selector/1 -> Data Store Write2/3  "<curVelNED>"
  Bus Assignment/1 -> Out1/1
  Bus Selector1/2 -> Data Type Conversion1/1  "<rolld>"
  input_euler_angle_roll_pitch_euler_rate_yaw4/8(pwm_tail_o) -> Bus Assignment/9  "pwm_tail"
  plane_mode_in/1 -> Data Store Write3/1
  input_euler_angle_roll_pitch_euler_rate_yaw4/6(tail_tilt_o) -> Bus Assignment/7  "tail_tilt"
  Data Type Conversion6/1 -> ?  "gyro_y"
  input_euler_angle_roll_pitch_euler_rate_yaw4/1(k_alieron_o) -> Bus Assignment/2  "k_aileron"
  CTRL_dbg_param/1 -> Data Store Write1/1
  Bus Selector3/1 -> Data Type Conversion3/1  "<airspeed_indicate>"
  Data Type Conversion/1 -> Data Store Write2/5  "pitchd"
  input_euler_angle_roll_pitch_euler_rate_yaw4/7(pwm_out_o) -> Bus Assignment/8  "pwm_out"
  Bus Selector3/2 -> Data Type Conversion4/1  "<EAS2TAS_Algo>"
  Bus Selector2/1 -> Data Type Conversion5/1  "<gyro_x>"
  Bus Selector1/3 -> Data Type Conversion2/1  "<yawd>"
  CTRL_wp/1 -> Data Store Write2/10  "wp_in"
  Data Type Conversion4/1 -> Data Store Write2/2  "EAS2TAS_Algo"
  Data Type Conversion3/1 -> Data Store Write2/1  "EAS_Algo"
  IMU/1 -> Bus Selector2/1
  PathModeOut/1 -> Data Store Write2/9  "PathModeOut"
  TASK_COMMON_OutParam/1 -> Bus Selector/1
  NAVI2CONTROL/1 -> Bus Selector1/1
  Bus Selector2/6 -> Data Type Conversion10/1  "<accel_z>"
  Bus Selector/2 -> Data Store Write2/4  "<curLLA>"
  Bus Selector2/4 -> Data Type Conversion8/1  "<accel_x>"
  EAS_Algo/1 -> Bus Selector3/1  "EAS_Algo"
  Data Type Conversion8/1 -> ?  "accel_x"
  Bus Selector2/5 -> Data Type Conversion9/1  "<accel_y>"
  CTRL_remote_ct_st/1 -> Data Store Write/1
  Bus Selector2/2 -> Data Type Conversion6/1  "<gyro_y>"
  Bus Selector2/3 -> Data Type Conversion7/1  "<gyro_z>"
  Constant/1 -> Bus Assignment/1
  Data Store Read2/1 -> Scope4/1
  Data Store Read3/1 -> Scope20/1
  Data Store Read15/1 -> Scope21/1
  Data Store Read16/1 -> MATLAB Function1/10(V)
  Add8/1 -> Gain/1
  Constant5/1 -> Subsystem/2(Density)
  MATLAB Function1/1(F) -> Add5/1
  Subsystem/1(Motor Forces) -> Scope23/1, Add5/2
  MATLAB Function1/2(M) -> Add7/1
  Subsystem/2(Motor Torques) -> Add7/2, Scope19/1
  Data Store Read17/1 -> Transpose/1, Scope17/1
  Constant2/1 -> Add8/2
  Gain/1 -> Sqrt/1
  Sqrt/1 -> Subsystem/4(Motor Commands)
  [Vb] -> Subsystem/1(Vb)
  [wb] -> Subsystem/3(pqr)
  Transpose/1 -> Add8/1
  Data Store Read18/1 -> Scope22/1
